simulink model "commander_old"  (R2024b)
settings: Solver=FixedStepAuto  StartTime=0.0  StopTime=100  FixedStep=0.5  RelTol=1e-3
(part 2 of 3)

== stateflow chart commander_old/Commander ==
  state initialize [parallel]
    en:
    commander_init();
    mission_init();
    led_init();
    buzzer_init();
    get_circuit_breaker_params();
    vehicle_type_init();
    arm_auth_init();
    note: 1. 后续删除commander_init()中的zero函数
  state parameters_update [parallel]
    en,du:
    com_params_update();
  state pre_flight_check [parallel]
    en,du:
    % 该模块对外输出变量boolean(preflight_check_res_)，true表示起飞检查通过；false表示起飞检查失败
    % report_failures_包括以下模块的错误
    report_failures_ = (report_failures_ && vehicle_status_flags_out_.condition_system_hotplug_timeout && ...
    ~vehicle_status_flags_out_.condition_calibration_enabled);
    % 初始化阶段（暂时写为1s）该模块不报错
    if uint64(getSimulationTime*1e+6) < 1e+6
    report_failures_ = false;
    prearm_ = true;
    end
    state airframeCheck [parallel]
    state sdcardCheck [parallel]
    state magCheck [parallel]
      en,du:
      if SYS_HAS_MAG == 1
      for i = 1:max_optional_mag_count
      % 第一个mag传感器是必要的
      required = boolean(bitshift(i-1, max_mandatory_mag_count));
      report_mag_fail = report_failures_;
      if ~magnetometerCheck(i, required, report_mag_fail)
      if required
      preflight_check_res_ = true;
      end
      report_mag_fail = false; % only report the first failure
      end
      end
      end
      % TODO: highest priority mag
      % mag consistency checks (need to be performed after the individual checks)
      if(~magConsistencyCheck(report_failures_))
      preflight_check_res_ = true;
      end
    state accelCheck [parallel]
      en,du:
      % check all sensors individually, but fail only for mandatory ones
      for i = 1:max_optional_accel_count
      required = boolean(bitshift(i-1, max_mandatory_mag_count));
      report_accel_fail = report_failures_;
      if(~accelerometerCheck(i, required, report_accel_fail) && required)
      preflight_check_res_ = true;
      end
      report_accel_fail = false; % only report the first failure
      end
    state gyroCheck [parallel]
      en,du:
      % check all sensors individually, but fail only for mandatory ones
      for i = 1:max_optional_gyro_count
      required = boolean(bitshift(i-1, max_optional_gyro_count));
      report_gyro_fail = report_failures_;
      if(~gyroCheck(i, required, report_gyro_fail) && required)
      preflight_check_res_ = true;
      end
      report_gyro_fail = false; % only report the first failure
      end
    state baroCheck [parallel]
      en,du:
      if SYS_HAS_BARO == true
      % check all sensors, but fail only for mandatory ones
      for i = 1:max_optional_baro_count
      required = boolean(bitshift(i-1, max_mandatory_mag_count));
      report_baro_fail = required && report_failures_;
      if(~baroCheck(i, required, report_baro_fail) && report_fail)
      report_baro_fail = true;
      end
      report_baro_fail = false; % only report the first failure
      end
      end
    state imuConsistencyCheck [parallel]
      en,du:
      % To be performed after the individual sensor checks have completed
      if ~imuConsistencyCheck(report_failures_)
      preflight_check_res_ = true;
      end
    state airspeedCheck [parallel]
      en,du:
      % Perform airspeed check only if circuit breaker is not engaged and it's not a rotary wing
      if ~vehicle_status_flags_out_.circuit_breaker_engaged_airspd_check && ...
      (vehicle_status_out_.vehicle_type == PX4_VEHICLE_STATUS.VEHICLE_TYPE_FIXED_WING || ...
      vehicle_status_out_.is_vtol)
      optional = (FW_ARSP_MODE == 1);
      airspeed_trim = FW_AIRSPD_TRIM;
      arming_max_airspeed_allowed = airspeed_trim / 2.0; % set to half of trim airspeed
      if (~airspeedCheck(optional, report_failures_, prearm_, COM_ARM_ARSP_EN, arming_max_airspeed_allowed) && ...
      ~optional)
      preflight_check_res_ = true;
      end
      end
    state rcCalibrationCheck [parallel]
      en,du:
      if vehicle_status_out_.rc_input_mode == PX4_VEHICLE_STATUS.RC_IN_MODE_DEFAULT
      if rcCheck(report_failures_, vehicle_status_out_.is_vtol)
      if report_failures_
      sprintf("mavlink_log_critical, RC calibration check failed");
      end
      preflight_check_res_ = true;
      set_health_flags(SUBSYSTEM_TYPE_RCRECEIVER, ...
      vehicle_status_flags_out_.rc_signal_found_once, ...
      true, ...
      false, ...
      vehicle_status_out_);
      else
      % The calibration is fine, but only set the overall health state to true if the signal is not currently lost
      vehicle_status_flags_out_.rc_calibration_valid = true;
      set_health_flags(SUBSYSTEM_TYPE_RCRECEIVER, ...
      vehicle_status_flags_out_.rc_signal_found_once, ...
      true, ...
      ~vehicle_status_out_.rc_signal_lost, ...
      vehicle_status_out_);
      end
      end
    state powerCheck [parallel]
      en,du:
      if vehicle_status_flags_out_.condition_power_input_valid && ...
      ~vehicle_status_flags_out_.circuit_breaker_engaged_power_check
      if ~powerCheck(report_failures_, prearm_)
      preflight_check_res_ = true;
      end
      end
    state failureDetectorCheck [parallel]
      en,du:
      if ~failureDetectorCheck(report_failures_)
      preflight_check_res_ = true;
      end
    state ekfCheck [parallel]
      en,du:
      % 仅支持EKF2，所以只检查EKF2
      ekf_healthy = ekf2Check(report_failures_) && ekf2CheckSensorBias(report_failures_);
      % For the first 10 seconds the ekf2 can be unhealthy, and we just mark it
      % as not present.
      % After that or if report_failures is true, we'll set the flags as is.
      time_since_boot = uint64(getSimulationTime*1e+6) - boot_timestamp_;
      if ~ekf_healthy && time_since_boot < 10*1e+6 && ~report_failures_
      set_health_flags(SUBSYSTEM_TYPE_AHRS, true, false, false, vehicle_status_out_);
      else
      set_health_flags(SUBSYSTEM_TYPE_AHRS, true, true, ekf_healthy, vehicle_status_out_);
      end
      preflight_check_res_ = preflight_check_res_ || ~ekf_healthy;
    state manualControlCheck [parallel]
      en,du:
      preflight_check_res_ = preflight_check_res_ || ~manualCheck(report_failures_);
    state cpuResourceCheck [parallel]
      en,du:
      preflight_check_res_ = preflight_check_res_ || ~cpuCheck(report_failures_);
  state topic_update [parallel]
    state offboard_update [parallel]
      en,du:
      % 预留
    state power_update [parallel]
      power_update -> (junction 4944) : [hasChanged(system_power.timestamp) && ...  (uint64(getSimulationTime*1e+6) - system_power.timestamp) < 1e+6]
      (junction 4944) -> (junction 4945) [order 1] : [system_power.servo_valid && ... ~system_power.brick_valid && ... ~system_power.usb_connected]
      (junction 4945) -> (junction 4946) : % 在只有舵机电源有效的情况下飞行，这是不安全的 {vehicle_status_flags_out_.condition_power_input_valid = false;}
      (junction 4944) -> (junction 4947) [order 2] : {vehicle_status_flags_out_.condition_power_input_valid = true;}
      (junction 4946) -> (junction 4948)
      (junction 4948) -> (junction 4947)
      (junction 4947) -> (junction 4949)
    state land_detector_update [parallel]
      en,du:
      % automatically set or update home position
      % set the home position when taking off, but only if we were previously disarmed
      % and at least 500 ms from commander start spent to avoid setting home on in-air restart
      if hasChanged(land_detector.timestamp) && actuator_armed.armed && ...
      ~home_position.manual_home && should_set_home_on_takeoff_ && land_detector_.landed && ...
      uint64(getSimulationTime*1e+6) > INAIR_RESTART_HOLDOFF_INTERVAL
      if was_landed
      should_set_home_on_takeoff_ = ~set_home_position();
      elseif COM_HOME_IN_AIR
      should_set_home_on_takeoff_ = ~set_in_air_home_position();
      end
      end
      % auto disarm after 5 seconds if kill switch is engaged
      if actuator_armed.armed && (actuator_armed.manual_lockdown || actuator_armed.lockdown)
      if elapsed(sec) > COM_KILL_DISARM && actuator_armed.manual_lockdown
      send(EVT_KILL_SWITCH, arming_state_transition);
      elseif elapsed(sec) > COM_KILL_DISARM
      send(EVT_LOCKDOWN, arming_state_transition);
      end
      end
      state land
        en:
        if uint64(getSimulationTime) ~= 0
        sprintf("mavlink_log_info: Landing detected");
        end
        vehicle_status_out_.takeoff_time = uint64(0);
        was_landed = land_detector.landed;
        du:
        % 在地面期间，有以下两种情况会自动上锁
        % 1. 着陆后，经过COM_DISARM_LAND秒后，无人机自动上锁；
        % 2. 解锁后，COM_DISARM_PRFLT秒内不起飞，无人机自动上锁；
        state situation1 [parallel]
          en,du:
          if (have_taken_off_since_arming_ && COM_DISARM_LAND > 0)
          if (elapsed(sec) > COM_DISARM_LAND)
          send(EVT_AUTO_DISARM_LAND, arming_state_transition);
          end
          end
        state situation2 [parallel]
          en,du:
          if (~have_taken_off_since_arming_ && COM_DISARM_PRFLT > 0)
          if (elapsed(sec) > COM_DISARM_PRFLT)
          send(EVT_AUTO_DISARM_PREFLIGHT, arming_state_transition);
          end
          end
      state takeoff
        en:
        sprintf("mavlink_log_info: Takeoff detected");
        vehicle_status_out_.takeoff_time = uint64(getSimulationTime*1e+6);
        have_taken_off_since_arming_ = true;
        was_landed = land_detector.landed;
        gpos_probation_time_us_ = COM_POS_FS_PROB*1e+6;
        lpos_probation_time_us_ = gpos_probation_time_us_;
        lvel_probation_time_us_ = gpos_probation_time_us_;
      (default) -> land
      land -> takeoff : [was_landed && ... ~land_detector.landed && ... actuator_armed.armed]
      takeoff -> land : [~was_landed && ... land_detector.landed && ... actuator_armed.armed]
    state safety_update [parallel]
      en,du:
      % 1. 没有解锁，安全开关没有按下去的时候，不允许解锁；
      % 2. 已经解锁，安全开关按下去，则加锁；
      if hasChanged(safety_switch.timestamp)
      set_health_flags(SUBSYSTEM_TYPE_MOTORCONTROL, ...
      safety_switch.safety_switch_available, ...
      safety_switch.safety_off, ...
      safety_switch.safety_switch_available, ....
      vehicle_status_out_);
      % disarm if safety is now on and still armed
      if actuator_armed_out_.armed && safety_switch.safety_switch_available && ~safety_switch.safety_off
      safety_disarm_allowed = (vehicle_status_out_.hil_state == PX4_VEHICLE_STATUS.HIL_STATE_OFF);
      % prevent disarming via safety button if not landed
      if (uint64(getSimulationTime*1e+6) - land_detector.timestamp) < 10*1e+6 && ~land_detector.landed
      safety_disarm_allowed = false;
      end
      if safety_disarm_allowed
      % disarm(arm_disarm_reason_t::SAFETY_BUTTON);
      send(EVT_SAFETY_BUTTON, arming_state_transition);
      end
      end
      end
      state safety_off
        en:
        g_status_changed = true;
        if uint64(getSimulationTime*1e+6) ~= 0
        % set_tune(tune_control_s::TUNE_ID_NOTIFY_POSITIVE);
        end
      state safety_on
        en:
        g_status_changed = true;
        % 闪烁白色LED，蜂鸣器neutral音调
        % tune_neutral(true);
        en,du:
        % 在着陆的状态下，才允许上锁
        if actuator_armed.armed && land_detector.landed
        send(EVT_DISARM, arming_state_transition);
        end
      (default) -> safety_off
      safety_off -> safety_on : [hasChanged(safety_switch.timestamp) && ... safety_switch.safety_switch_available && ... ~safety_switch.safety_off]
      safety_on -> safety_off : [hasChanged(safety_switch.timestamp) && ... safety_switch.safety_switch_available && ... safety_switch.safety_off]
    state vtol_status_update [parallel]
      en,du:
      if hasChanged(vtol_status.timestamp)
      update_vtol_status();
      end
    state esc_status_update [parallel]
      en,du:
      if hasChanged(esc_status.timestamp)
      last_esc_status_updated = esc_status_check();
      elseif COM_ARM_CHK_ESCS ~= 0 && ~vehicle_status_flags_out_.condition_escs_error
      if (last_esc_status_updated ~= 0) && (uint64(getSimulationTime*1e+6 - last_esc_status_updated) > 700*1e+3)
      % Detect timeout after first telemetry packet received
      % Some DShot ESCs are unresponsive for ~550ms during their initialization, so we use a timeout higher than that
      sprintf("mavlink_log_critical, ESCs telemetry timeout");
      vehicle_status_flags_out_.condition_escs_error = true;
      elseif (last_esc_status_updated == 0) && (uint64(getSimulationTime*1e+6 - boot_timestamp_) > 5*1e+6)
      % Detect if esc telemetry is not connected after reboot
      sprintf("mavlink_log_critical, ESCs telemetry not connected ");
      vehicle_status_flags_out_.condition_escs_error = true;
      end
      end
    state estimator_check [parallel]
      en,du:
      ekf_status_check();
    state battery_status_check [parallel]
      battery_status_check -> (junction 4987) : % execute battery failsafe if the state has gotten worse while we are armed {[battery_warning, battery_warning_level_increased_while_armed] = battery_check();}
      (junction 4987) -> (junction 4988) : [battery_warning_level_increased_while_armed]
      (junction 4988) -> (junction 4989) [order 1] : [battery_warning == uint8(PX4_BATTERY_STATUS.BATTERY_WARNING_NONE)]
      (junction 4988) -> (junction 4990) [order 2]
      (junction 4989) -> (junction 5003)
      (junction 4990) -> (junction 4991) [order 1] : [battery_warning == uint8(PX4_BATTERY_STATUS.BATTERY_WARNING_LOW)]
      (junction 4990) -> (junction 4992) [order 2]
      (junction 4991) -> (junction 5002) : {sprintf("mavlink_log_critical, Low battery level! Return advised");}
      (junction 4992) -> (junction 4993) [order 1] : [battery_warning == uint8(PX4_BATTERY_STATUS.BATTERY_WARNING_CRITICAL)]
      (junction 4992) -> (junction 4994) [order 2]
      (junction 4993) -> (junction 5001) : {battery_warning_critical();}
      (junction 4994) -> (junction 4995) [order 1] : [battery_warning == uint8(PX4_BATTERY_STATUS.BATTERY_WARNING_EMERGENCY)]
      (junction 4994) -> (junction 4996) [order 2]
      (junction 4995) -> (junction 5000) : {battery_warning_emergency();}
      (junction 4996) -> (junction 4997) [order 1] : [battery_warning == uint8(PX4_BATTERY_STATUS.BATTERY_WARNING_FAILED)]
      (junction 4996) -> (junction 4998) [order 2]
      (junction 4997) -> (junction 4999) : {sprintf("mavlink_log_emergency, Battery failure detected");}
      (junction 4999) -> (junction 4998)
      (junction 5000) -> (junction 4999)
      (junction 5001) -> (junction 5000)
      (junction 5002) -> (junction 5001)
      (junction 5003) -> (junction 5002)
      (junction 4998) -> (junction 5004)
    state mission_result_update [parallel]
      en:
      % start mission result check
      if hasChanged(mission_result.timestamp)
      evaluate_mission_state();
      end
      % Transition main state to loiter or auto-mission after takeoff is completed.
      if actuator_armed.armed && ~land_detector.landed && ...
      (vehicle_status_out_.nav_state == uint8(PX4_VEHICLE_STATUS.NAVIGATION_STATE_AUTO_TAKEOFF)) && ...
      (mission_result.timestamp >= vehicle_status_out_.nav_state_timestamp) && ...
      mission_result.finished
      if COM_TAKEOFF_ACT == 1  && vehicle_status_flags_out_.condition_auto_mission_available
      main_state_transition(PX4_COMMANDER_STATE.MAIN_STATE_AUTO_MISSION);
      else
      main_state_transition(PX4_COMMANDER_STATE.MAIN_STATE_AUTO_LOITER);
      end
      end
    state geofence_update [parallel]
      en,du:
      % start geofence result check
      vehicle_status_out_.geofence_violated = geofence_result.geofence_violated;
      geofence_check();
    state check_mission_flight_termination [parallel]
      en,du:
      if actuator_armed.armed && mission_result.flight_termination && ...
      ~vehicle_status_flags_out_.circuit_breaker_flight_termination_disabled
      % send_parachute_command();
      g_status_changed = true;
      actuator_armed_out_.force_failsafe = true;
      sprintf("mavlink_log_critical, Geofence violation! Flight terminated");
      if every(500, tick)
      sprintf("mavlink_log_critical, Flight termination active")
      end
      end
    state manual_control_update [parallel]
      en,du:
      manual_control_input_handling();
    state data_link_check [parallel]
    state avoidance_check [parallel]
    state check_arming_state_change [parallel]
      check_arming_state_change -> (junction 6796)
      (junction 6796) -> (junction 6797) [order 1] : [was_armed ~= actuator_armed.armed]
      (junction 6797) -> (junction 6798) : {g_status_changed = true;}
      (junction 6798) -> (junction 6799) [order 1] : [actuator_armed.armed && ~land_detector.landed]
      (junction 6799) -> (junction 6800) : % check if takeoff already detected upon arming {have_taken_off_since_arming_ = true;}
      (junction 6796) -> (junction 6803) [order 2]
      (junction 6798) -> (junction 6801) [order 2]
      (junction 6800) -> (junction 6802)
      (junction 6801) -> (junction 6802) : % increase the flight uuid upon disarming % flight_uuid = _param_flight_uuid.get() + 1;  % param_flight_uuid.set(flight_uuid); % param_flight_uuid.commit_no_notification();] {last_disarmed_timestamp_ = uint64(getSimulationTime * 1e+6); should_set_home_on_takeoff_ = true;}
      (junction 6802) -> (junction 6804)
      (junction 6804) -> (junction 6803)
      (junction 6803) -> (junction 6805)
      (junction 6805) -> (junction 6806) [order 1] : % Reset the flag if disarmed [actuator_armed.armed]
      (junction 6806) -> (junction 6807) : {have_taken_off_since_arming_ = false;}
      (junction 6805) -> (junction 6808) [order 2]
      (junction 6807) -> (junction 6809)
      (junction 6809) -> (junction 6808)
      (junction 6808) -> (junction 6810) : {was_armed = actuator_armed.armed;}
    state actuator_control_update [parallel]
      % engine failure detection
      % TODO: move out of commander
      actuator_control_update -> (junction 5052) : [hasChanged(actuator_controls.timestamp)]
      (junction 5052) -> (junction 5053) [order 1] : [~vehicle_status_flags_out_.circuit_breaker_engaged_enginefailure_check && ... vehicle_status_out_.vehicle_type == uint8(PX4_VEHICLE_STATUS.VEHICLE_TYPE_FIXED_WING) && ... ~vehicle_status_out_.is_vtol && actuator_armed.armed]
      (junction 5052) -> (junction 5054) [order 2] : {reset_failure_flags();}
      (junction 5053) -> (junction 5055) : {check_engine_failure_for_fixed_wing();}
      (junction 5055) -> (junction 5054)
      (junction 5054) -> (junction 5056)
    state tablet_control_update [parallel]
      en,du:
      % 平板控制
    state home_position_update [parallel]
      % automatically set or update home position
      home_position_update -> (junction 6370) : [~home_position.manual_home && ... ~actuator_armed.armed]
      (junction 6370) -> (junction 6371) [order 1] : % 未解锁，飞机着陆，没有手动设置home点，local_pos有效 [home_position.valid_lpos && ... land_detector.landed && ...  local_position.xy_valid && ... local_position.z_valid]
      (junction 6371) -> (junction 6372) : {set_home_lpos_valid();}
      (junction 6370) -> (junction 6373) [order 2] : {set_home_lpos_invalid();}
      (junction 6372) -> (junction 6374)
      (junction 6374) -> (junction 6373)
      (junction 6373) -> (junction 6375)
  state commands_update [parallel]
    % request to set different system mode
    state DO_REPOSITION [parallel]
      DO_REPOSITION -> (junction 5069) : [hasChanged(cmd.timestamp) && ... cmd.command == PX4_VEHICLE_COMMAND.VEHICLE_CMD_DO_REPOSITION]
      (junction 5069) -> (junction 5070) [order 1] : % Check if a mode switch had been requested [bitget(uint32(cmd.param2), 1) > 0]
      (junction 5070) -> (junction 5071) [order 1] : [main_state_transition(PX4_COMMANDER_STATE.MAIN_STATE_AUTO_LOITER) ~= TRANSITION_DENIED]
      (junction 5069) -> (junction 5072) [order 2] : {g_status_changed = true;}
      (junction 5070) -> (junction 5073) [order 2] : {g_status_changed = false;  sprintf("mavlink_log_critical, Reposition command rejected")}
      (junction 5071) -> (junction 5074) : {g_status_changed = true;}
      (junction 5073) -> (junction 5072)
      (junction 5074) -> (junction 5073)
      (junction 5072) -> (junction 5075)
    state DO_SET_MODE [parallel]
      note: VEHICLE_MODE_FLAG_CUSTOM_MODE_ENABLED = 1, /* 0b00000001 Reserved for future use. | */ VEHICLE_MODE_FLAG_TEST_ENABLED = 2, /* 0b00000010 system has a test mode enabled. This flag is intended for temporary system tests and should not be used for stable implementations. | */ VEHICLE_MODE_FLAG_AUTO_ENABLED = 4, /* 0b00000100 autonomous mode enabled, system finds its own goal positions. Guided flag can be set or not, depends on the actual implementation. | */ VEHICLE_MODE_FLAG_GUIDED_ENABLED = 8, /* 0b00001000 guided mode enabled, system flies MISSIONs / mission items. | */ VEHICLE_MODE_FLAG_STABILIZE_ENABLED = 16, /* 0b00010000 system stabilizes electronically its attitude (and optionally position). It needs however further control inputs to move around. | */ VEHICLE_MODE_FLAG_HIL_ENABLED = 32, /* 0b00100000 hardware in the loop simulation. All motors / actuators are blocked, but internal software is full operational. | */ VEHICLE_MODE_FLAG_MANUAL_INPUT_ENABLED = 64, /* 0b01000000 remote control input is enabled. | */ VEHICLE_MODE_FLAG_SAFETY_ARMED = 128, /* 0b10000000 MAV safety set to armed. Motors are enabled / running / can start. Ready to fly. Additional note: this flag is to be ignore when sent in the command MAV_CMD_DO_SET_MODE and MAV_CMD_COMPONENT_ARM_DISARM shall be used instead. The flag can still be used to report the armed state. | */ VEHICLE_MODE_FLAG_ENUM_END = 129, /* | */
      DO_SET_MODE -> (junction 5090) : [hasChanged(cmd.timestamp) && ... cmd.command == PX4_VEHICLE_COMMAND.VEHICLE_CMD_DO_SET_MODE]
      (junction 5090) -> (junction 5091) : % action {base_mode = uint8(cmd.param1); custom_main_mode = uint8(cmd.param2); custom_sub_mode = uint8(cmd.param3);}
      (junction 5091) -> (junction 5092) [order 1] : % custom mode enable [bitand(base_mode, VEHICLE_MODE_FLAG_CUSTOM_MODE_ENABLED)]
      (junction 5092) -> (junction 5093) [order 1] : [custom_main_mode == PX4_CUSTOM_MAIN_MODE.MANUAL]
      (junction 5093) -> (junction 5094) : {new_main_state = uint8(PX4_COMMANDER_STATE.MAIN_STATE_MANUAL);}
      (junction 5091) -> (junction 5139) [order 2]
      (junction 5092) -> (junction 5095) [order 2]
      (junction 5094) -> (junction 5097)
      (junction 5095) -> (junction 5096) [order 1] : [custom_main_mode == PX4_CUSTOM_MAIN_MODE.ALTCTL]
      (junction 5096) -> (junction 5097) : {new_main_state = uint8(PX4_COMMANDER_STATE.MAIN_STATE_ALTCTL);}
      (junction 5095) -> (junction 5098) [order 2]
      (junction 5097) -> (junction 5100)
      (junction 5098) -> (junction 5099) [order 1] : [custom_main_mode == PX4_CUSTOM_MAIN_MODE.POSCTL]
      (junction 5099) -> (junction 5100) : {reset_posvel_validity(); new_main_state = uint8(PX4_COMMANDER_STATE.MAIN_STATE_POSCTL);}
      (junction 5098) -> (junction 5101) [order 2]
      (junction 5100) -> (junction 5104)
      (junction 5101) -> (junction 5102) [order 1] : [custom_main_mode == PX4_CUSTOM_MAIN_MODE.AUTO] {reset_posvel_validity();}
      (junction 5102) -> (junction 5103) [order 1] : [custom_sub_mode == PX4_CUSTOM_SUB_MODE_AUTO.LOITER]
      (junction 5103) -> (junction 5104) : {new_main_state = uint8(PX4_COMMANDER_STATE.MAIN_STATE_AUTO_LOITER);}
      (junction 5101) -> (junction 5128) [order 2]
      (junction 5102) -> (junction 5105) [order 2]
      (junction 5104) -> (junction 5107)
      (junction 5105) -> (junction 5106) [order 1] : [custom_sub_mode == PX4_CUSTOM_SUB_MODE_AUTO.MISSION]
      (junction 5106) -> (junction 5107) : {new_main_state = uint8(PX4_COMMANDER_STATE.MAIN_STATE_AUTO_MISSION);}
      (junction 5105) -> (junction 5108) [order 2]
      (junction 5107) -> (junction 5110)
      (junction 5108) -> (junction 5109) [order 1] : [custom_sub_mode == PX4_CUSTOM_SUB_MODE_AUTO.RTL]
      (junction 5109) -> (junction 5110) : {new_main_state = uint8(PX4_COMMANDER_STATE.MAIN_STATE_AUTO_RTL);}
      (junction 5108) -> (junction 5111) [order 2]
      (junction 5110) -> (junction 5113)
      (junction 5111) -> (junction 5112) [order 1] : [custom_sub_mode == PX4_CUSTOM_SUB_MODE_AUTO.TAKEOFF]
      (junction 5112) -> (junction 5113) : {new_main_state = uint8(PX4_COMMANDER_STATE.MAIN_STATE_AUTO_TAKEOFF);}
      (junction 5111) -> (junction 5114) [order 2]
      (junction 5113) -> (junction 5116)
      (junction 5114) -> (junction 5115) [order 1] : [custom_sub_mode == PX4_CUSTOM_SUB_MODE_AUTO.LAND]
      (junction 5115) -> (junction 5116) : {new_main_state = uint8(PX4_COMMANDER_STATE.MAIN_STATE_AUTO_LAND);}
      (junction 5114) -> (junction 5117) [order 2]
      (junction 5116) -> (junction 5119)
      (junction 5117) -> (junction 5118) [order 1] : [custom_sub_mode == PX4_CUSTOM_SUB_MODE_AUTO.FOLLOW_TARGET]
      (junction 5118) -> (junction 5119) : {new_main_state = uint8(PX4_COMMANDER_STATE.MAIN_STATE_AUTO_FOLLOW_TARGET);}
      (junction 5117) -> (junction 5120) [order 2]
      (junction 5119) -> (junction 5122)
      (junction 5120) -> (junction 5121) [order 1] : [custom_sub_mode == PX4_CUSTOM_SUB_MODE_AUTO.PRECLAND]
      (junction 5121) -> (junction 5122) : {new_main_state = uint8(PX4_COMMANDER_STATE.MAIN_STATE_AUTO_PRECLAND);}
      (junction 5120) -> (junction 5123) [order 2]
      (junction 5122) -> (junction 5125)
      (junction 5123) -> (junction 5124) [order 1] : [custom_sub_mode > 0]
      (junction 5124) -> (junction 5125) : {sprintf("mavlink_log_critical, Unsupported auto mode") new_main_state = uint8(PX4_COMMANDER_STATE.MAIN_STATE_MAX);}
      (junction 5123) -> (junction 5126) [order 2]
      (junction 5125) -> (junction 5127)
      (junction 5126) -> (junction 5127) : {new_main_state = uint8(PX4_COMMANDER_STATE.MAIN_STATE_AUTO_MISSION);}
      (junction 5128) -> (junction 5129) [order 1] : [custom_main_mode == PX4_CUSTOM_MAIN_MODE.ACRO]
      (junction 5129) -> (junction 5130) : {new_main_state = uint8(PX4_COMMANDER_STATE.MAIN_STATE_ACRO);}
      (junction 5128) -> (junction 5131) [order 2]
      (junction 5130) -> (junction 5133)
      (junction 5131) -> (junction 5132) [order 1] : [custom_main_mode == PX4_CUSTOM_MAIN_MODE.STABILIZED]
      (junction 5132) -> (junction 5133) : {new_main_state = uint8(PX4_COMMANDER_STATE.MAIN_STATE_STAB);}
      (junction 5131) -> (junction 5134) [order 2]
      (junction 5133) -> (junction 5136)
      (junction 5134) -> (junction 5135) [order 1] : [custom_main_mode == PX4_CUSTOM_MAIN_MODE.OFFBOARD]
      (junction 5135) -> (junction 5136) : {reset_posvel_validity(); new_main_state = uint8(PX4_COMMANDER_STATE.MAIN_STATE_OFFBOARD);}
      (junction 5134) -> (junction 5137) [order 2]
      (junction 5136) -> (junction 5138)
      (junction 5137) -> (junction 5138) : {new_main_state = uint8(PX4_COMMANDER_STATE.MAIN_STATE_MAX);}
      (junction 5138) -> (junction 5141)
      (junction 5139) -> (junction 5140) [order 1] : % AUTO_MODE_ENABLE [bitand(base_mode, VEHICLE_MODE_FLAG_AUTO_ENABLED)]
      (junction 5140) -> (junction 5141) : {new_main_state = uint8(PX4_COMMANDER_STATE.MAIN_STATE_AUTO_MISSION);}
      (junction 5139) -> (junction 5142) [order 2]
      (junction 5141) -> (junction 5145)
      (junction 5142) -> (junction 5143) [order 1] : [bitand(base_mode, VEHICLE_MODE_FLAG_MANUAL_INPUT_ENABLED)]
      (junction 5143) -> (junction 5144) [order 1] : [bitand(base_mode, VEHICLE_MODE_FLAG_GUIDED_ENABLED)]
      (junction 5144) -> (junction 5145) : {new_main_state = uint8(PX4_COMMANDER_STATE.MAIN_STATE_POSCTL);}
      (junction 5142) -> (junction 5151) [order 2]
      (junction 5143) -> (junction 5146) [order 2]
      (junction 5145) -> (junction 5148)
      (junction 5146) -> (junction 5147) [order 1] : [bitand(base_mode, VEHICLE_MODE_FLAG_STABILIZE_ENABLED)]
      (junction 5147) -> (junction 5148) : {new_main_state = uint8(PX4_COMMANDER_STATE.MAIN_STATE_STAB);}
      (junction 5146) -> (junction 5149) [order 2]
      (junction 5148) -> (junction 5150)
      (junction 5149) -> (junction 5150) : {new_main_state = uint8(PX4_COMMANDER_STATE.MAIN_STATE_MANUAL);}
      (junction 5150) -> (junction 5152)
      (junction 5152) -> (junction 5151)
      (junction 5151) -> (junction 5153) : {main_state_transition(new_main_state);}
    state COMPONENT_ARM_DISARM [parallel]
      COMPONENT_ARM_DISARM -> (junction 5253) : [hasChanged(cmd.timestamp) && ... cmd.command == PX4_VEHICLE_COMMAND.VEHICLE_CMD_COMPONENT_ARM_DISARM]
      (junction 5253) -> (junction 5254) : {param1_arm = round(cmd.param1);}
      (junction 5254) -> (junction 5255) [order 1] : [param1_arm ~= 0 && param1_arm ~= 1]{sprintf("mavlink_log_critical, Unsupported ARM_DISARM param")}
      (junction 5254) -> (junction 5256) [order 2] : % Arm is forced (checks skipped) when param2 is set to a magic number. {cmd_arms = (param1_arm == 1);  force = round(cmd.param2) == 21196;}
      (junction 5255) -> (junction 5286)
      (junction 5257) -> (junction 5258) [order 1] : [~(land_detector.landed || land_detector.maybe_landed) && ...  ~is_ground_rover(vehicle_status_out_) ]
      (junction 5258) -> (junction 5259) [order 1] : [cmd_arms]
      (junction 5259) -> (junction 5260) [order 1] : [actuator_armed.armed]
      (junction 5256) -> (junction 5257) [order 1] : [~force]
      (junction 5256) -> (junction 5274) [order 2]
      (junction 5257) -> (junction 5261) [order 2]
      (junction 5258) -> (junction 5262) [order 2] : {sprintf("mavlink_log_critical, Disarming denied! Not landed")}
      (junction 5259) -> (junction 5263) [order 2] : {sprintf("mavlink_log_critical, Arming denied! Not landed")}
      (junction 5260) -> (junction 5264) : {sprintf("mavlink_log_warning, Arming denied! Already armed")}
      (junction 5262) -> (junction 5261)
      (junction 5263) -> (junction 5262)
      (junction 5264) -> (junction 5263)
      (junction 5261) -> (junction 5265) : {cmd_from_io = round(cmd.param3) == 1234;}
      (junction 5265) -> (junction 5266) [order 1] : % Flick to in-air restore first if this comes from an onboard system and from IO [cmd.source_system == vehicle_status_out_.system_id && ...  cmd.source_component == vehicle_status_out_.component_id && ...  cmd_from_io && cmd_arms]
      (junction 5265) -> (junction 5267) [order 2]
      (junction 5266) -> (junction 5268)
      (junction 5268) -> (junction 5267) : {vehicle_status_out_.arming_state = uint8(PX4_VEHICLE_STATUS.ARMING_STATE_IN_AIR_RESTORE);}
      (junction 5267) -> (junction 5269)
      (junction 5269) -> (junction 5270) [order 1] : [cmd_arms]
      (junction 5270) -> (junction 5271) [order 1] : [cmd.from_external]
      (junction 5269) -> (junction 5272) [order 2]
      (junction 5270) -> (junction 5277) [order 2] : %{arm(COMMAND_INTERNAL, ~forced);}
      (junction 5271) -> (junction 5278) : %{arming_res = arm(COMMAND_EXTERNAL);}
      (junction 5272) -> (junction 5273) [order 1] : [cmd.from_external]
      (junction 5272) -> (junction 5275) [order 2] : %{disarm(COMMAND_INTERNAL);}
      (junction 5273) -> (junction 5276) : %{disarm(COMMAND_EXTERNAL);}
      (junction 5275) -> (junction 5274)
      (junction 5277) -> (junction 5276)
      (junction 5278) -> (junction 5277)
      (junction 5276) -> (junction 5275)
      (junction 5274) -> (junction 5279)
      (junction 5279) -> (junction 5280) [commented out] : [arming_res == TRANSITION_DENIED]
      (junction 5279) -> (junction 5281)
      (junction 5280) -> (junction 5285) [commented out]
      (junction 5281) -> (junction 5282) [commented out] : [cmd_arms && (arming_res == TRANSITION_CHANGED) && (hrt_absolute_time() > (_boot_timestamp + INAIR_RESTART_HOLDOFF_INTERVAL)) && ~_home_pub.get().manual_home]
      (junction 5281) -> (junction 5283)
      (junction 5282) -> (junction 5284) [commented out] : {set_home_position();}
      (junction 5284) -> (junction 5283)
      (junction 5285) -> (junction 5284)
      (junction 5286) -> (junction 5285)
      (junction 5283) -> (junction 5287)
    state FLIGHTTERMINATION [parallel]
      FLIGHTTERMINATION -> (junction 5335) : [hasChanged(cmd.timestamp) && ... cmd.command == PX4_VEHICLE_COMMAND.VEHICLE_CMD_DO_FLIGHTTERMINATION]
      (junction 5335) -> (junction 5336) [order 1] : [cmd.param1 > 1.5 && ~lockdown_triggered_]
      (junction 5336) -> (junction 5337) : {actuator_armed_out_.lockdown = true; lockdown_triggered_ = true; sprintf("PX4_WARN, forcing lockdown (motors off)")}
      (junction 5335) -> (junction 5338) [order 2]
      (junction 5337) -> (junction 5341)
      (junction 5339) -> (junction 5340) [order 1] : [~flight_termination_triggered_]
      (junction 5338) -> (junction 5339) [order 1] : [cmd.param1 > 0.5]
      (junction 5340) -> (junction 5341) : {actuator_armed_out_.force_failsafe = true; flight_termination_triggered_ = true; sprintf("PX4_WARN, forcing failsafe (termination)")}
      (junction 5338) -> (junction 5345) [order 2] : {actuator_armed_out_.force_failsafe = true; actuator_armed_out_.lockdown = false; lockdown_triggered_ = false; flight_termination_triggered_ = false; sprintf("PX4_WARN, disabling failsafe and lockdown")}
      (junction 5339) -> (junction 5342) [order 2]
      (junction 5341) -> (junction 5344)
      (junction 5342) -> (junction 5343) : [uint8(cmd.param2) < 0]
      (junction 5343) -> (junction 5344) : {sprintf("PX4_WARN, reset all non-flighttermination failsafe commands")}
      (junction 5344) -> (junction 5346)
      (junction 5346) -> (junction 5345)
      (junction 5345) -> (junction 5347) : {cmd_result_ = uint8(PX4_VEHICLE_COMMAND.VEHICLE_CMD_RESULT_ACCEPTED)}
    state SET_HOME [parallel]
      SET_HOME -> (junction 5369) : [hasChanged(cmd.timestamp) && ... cmd.command == PX4_VEHICLE_COMMAND.VEHICLE_CMD_DO_SET_HOME]
      (junction 5369) -> (junction 5370) : {use_current = (cmd.param1 > 0.5);}
      (junction 5372) -> (junction 5373) : {cmd_result_ == uint8(PX4_VEHICLE_COMMAND.VEHICLE_CMD_RESULT_ACCEPTED);}
      (junction 5370) -> (junction 5371) [order 1] : [use_current]
      (junction 5371) -> (junction 5372) [order 1] : [set_home_position()]
      (junction 5370) -> (junction 5376) [order 2] : {lat = cmd.param5; lon = cmd.param6; alt = cmd.param7;}
      (junction 5371) -> (junction 5374) [order 2]
      (junction 5373) -> (junction 5375)
      (junction 5374) -> (junction 5375) : {cmd_result_ == uint8(PX4_VEHICLE_COMMAND.VEHICLE_CMD_RESULT_TEMPORARILY_REJECTED);}
      (junction 5375) -> (junction 5378)
      (junction 5376) -> (junction 5377) [order 1] : % 自定义home点位置 [isfinite(lat) && isfinite(lon) && isfinite(alt)]
      (junction 5377) -> (junction 5378) : {set_custom_home_position(lat, lon, alt);}
      (junction 5376) -> (junction 5379) [order 2] : {cmd_result_ == uint8(PX4_VEHICLE_COMMAND.VEHICLE_CMD_RESULT_DENIED);}
      (junction 5378) -> (junction 5380)
      (junction 5380) -> (junction 5379)
      (junction 5379) -> (junction 5381)
    state NAV_RETURN_TO_LAUNCH [parallel]
      NAV_RETURN_TO_LAUNCH -> (junction 5403) : [hasChanged(cmd.timestamp) && ... cmd.command == PX4_VEHICLE_COMMAND.VEHICLE_CMD_NAV_RETURN_TO_LAUNCH]
      (junction 5403) -> (junction 5404) [order 1] : [main_state_transition(PX4_COMMANDER_STATE.MAIN_STATE_AUTO_LOITER) == TRANSITION_CHANGED]
      (junction 5404) -> (junction 5405) : {sprintf("mavlink_log_critical, Returning to launch") cmd_result_ == uint8(PX4_VEHICLE_COMMAND.VEHICLE_CMD_RESULT_ACCEPTED);}
      (junction 5403) -> (junction 5406) [order 2] : {sprintf("mavlink_log_critical, Return to launch denied") cmd_result_ == uint8(PX4_VEHICLE_COMMAND.VEHICLE_CMD_RESULT_TEMPORARILY_REJECTED);}
      (junction 5405) -> (junction 5407)
      (junction 5407) -> (junction 5406)
      (junction 5406) -> (junction 5408)
    state NAV_TAKEOFF [parallel]
      NAV_TAKEOFF -> (junction 5417) : [hasChanged(cmd.timestamp) && ... cmd.command == PX4_VEHICLE_COMMAND.VEHICLE_CMD_NAV_TAKEOFF]
      (junction 5418) -> (junction 5419) : {cmd_result_ == uint8(PX4_VEHICLE_COMMAND.VEHICLE_CMD_RESULT_ACCEPTED);}
      (junction 5417) -> (junction 5418) [order 1] : [main_state_transition(PX4_COMMANDER_STATE.MAIN_STATE_AUTO_TAKEOFF) == TRANSITION_CHANGED]
      (junction 5417) -> (junction 5420) [order 2]
      (junction 5419) -> (junction 5422)
      (junction 5420) -> (junction 5421) [order 1] : [internal_state_out_.main_state == PX4_COMMANDER_STATE.MAIN_STATE_AUTO_TAKEOFF]
      (junction 5421) -> (junction 5422) : {cmd_result_ == uint8(PX4_VEHICLE_COMMAND.VEHICLE_CMD_RESULT_ACCEPTED);}
      (junction 5420) -> (junction 5423) [order 2] : {cmd_result_ == uint8(PX4_VEHICLE_COMMAND.VEHICLE_CMD_RESULT_TEMPORARILY_REJECTED);}
      (junction 5422) -> (junction 5424)
      (junction 5424) -> (junction 5423)
      (junction 5423) -> (junction 5425)
    state NAV_LAND [parallel]
      NAV_LAND -> (junction 5438) : [hasChanged(cmd.timestamp) && ... cmd.command == PX4_VEHICLE_COMMAND.VEHICLE_CMD_NAV_LAND]
      (junction 5438) -> (junction 5439) [order 1] : [main_state_transition(PX4_COMMANDER_STATE.MAIN_STATE_AUTO_LAND) ~= TRANSITION_DENIED]
      (junction 5439) -> (junction 5440) : {sprintf("mavlink_log_info, Landing at current position") cmd_result_ == uint8(PX4_VEHICLE_COMMAND.VEHICLE_CMD_RESULT_ACCEPTED);}
      (junction 5438) -> (junction 5441) [order 2] : {sprintf("mavlink_log_critical, Landing denied! Please land manually") cmd_result_ == uint8(PX4_VEHICLE_COMMAND.VEHICLE_CMD_RESULT_TEMPORARILY_REJECTED);}
      (junction 5440) -> (junction 5442)
      (junction 5442) -> (junction 5441)
      (junction 5441) -> (junction 5443)
    state NAV_PRECLAND [parallel]
      NAV_PRECLAND -> (junction 5452) : [hasChanged(cmd.timestamp) && ... cmd.command == PX4_VEHICLE_COMMAND.VEHICLE_CMD_NAV_PRECLAND]
      (junction 5453) -> (junction 5454) : {sprintf("mavlink_log_info, Precision landing") cmd_result_ == uint8(PX4_VEHICLE_COMMAND.VEHICLE_CMD_RESULT_ACCEPTED);}
      (junction 5452) -> (junction 5453) [order 1] : [main_state_transition(PX4_COMMANDER_STATE.MAIN_STATE_AUTO_PRECLAND) ~= TRANSITION_DENIED]
      (junction 5452) -> (junction 5455) [order 2] : {sprintf("mavlink_log_critical, Precision landing denied! Please land manually") cmd_result_ == uint8(PX4_VEHICLE_COMMAND.VEHICLE_CMD_RESULT_TEMPORARILY_REJECTED);}
      (junction 5454) -> (junction 5456)
      (junction 5456) -> (junction 5455)
      (junction 5455) -> (junction 5457)
    state MISSION_START [parallel]
      MISSION_START -> (junction 5466) : [hasChanged(cmd.timestamp) && ... cmd.command == PX4_VEHICLE_COMMAND.VEHICLE_CMD_MISSION_START]
      (junction 5466) -> (junction 5467) [order 1] : [vehicle_status_flags_out_.condition_auto_mission_available]
      (junction 5467) -> (junction 5468) : [isfinite(cmd.param1) && isfinite(cmd.param1 >= -1) && ... cmd.param1 < mission_result.seq_total]
      (junction 5468) -> (junction 5469) [order 1] : % 条件没写完 [main_state_transition(PX4_COMMANDER_STATE.MAIN_STATE_AUTO_MISSION) ~= TRANSITION_DENIED]
      (junction 5469) -> (junction 5470) : {cmd_result_ == uint8(PX4_VEHICLE_COMMAND.VEHICLE_CMD_RESULT_ACCEPTED);}
      (junction 5466) -> (junction 5471) [order 2] : {sprintf("mavlink_log_critical, Mission start denied! No valid mission") cmd_result_ == uint8(PX4_VEHICLE_COMMAND.VEHICLE_CMD_RESULT_DENIED);}
      (junction 5468) -> (junction 5472) [order 2] : {sprintf("mavlink_log_critical, Mission start denied") cmd_result_ == uint8(PX4_VEHICLE_COMMAND.VEHICLE_CMD_RESULT_TEMPORARILY_REJECTED);}
      (junction 5470) -> (junction 5473)
      (junction 5472) -> (junction 5471)
      (junction 5473) -> (junction 5472)
      (junction 5471) -> (junction 5474)
    state HIGH_LATENCY [parallel]
      HIGH_LATENCY -> (junction 5487) : [hasChanged(cmd.timestamp) && ... cmd.command == PX4_VEHICLE_COMMAND.VEHICLE_CMD_CONTROL_HIGH_LATENCY]
      (junction 5488) -> (junction 5489) : % if no high latency telemetry exists send a failed acknowledge {sprintf("mavlink_log_critical, Control high latency failed! Telemetry unavailable") cmd_result_ = uint8(PX4_VEHICLE_COMMAND.VEHICLE_CMD_RESULT_FAILED);}
      (junction 5487) -> (junction 5488) [order 1] : [high_latency_datalink_heartbeat_ > boot_timestamp_]
      (junction 5487) -> (junction 5490) [order 2]
      (junction 5489) -> (junction 5491)
      (junction 5491) -> (junction 5490)
      (junction 5490) -> (junction 5492)
    state ORBIT [parallel]
      ORBIT -> (junction 5501) : [hasChanged(cmd.timestamp) && ... cmd.command == PX4_VEHICLE_COMMAND.VEHICLE_CMD_DO_ORBIT]
      (junction 5501) -> (junction 5502) [order 1] : [main_state_transition(PX4_COMMANDER_STATE.MAIN_STATE_ORBIT) ~= TRANSITION_DENIED]
      (junction 5502) -> (junction 5503) : {cmd_result_ == uint8(PX4_VEHICLE_COMMAND.VEHICLE_CMD_RESULT_ACCEPTED);}
      (junction 5503) -> (junction 5505)
      (junction 5501) -> (junction 5504) [order 2] : {cmd_result_ == uint8(PX4_VEHICLE_COMMAND.VEHICLE_CMD_RESULT_TEMPORARILY_REJECTED);}
      (junction 5505) -> (junction 5504)
      (junction 5504) -> (junction 5506)
    state TEST_MOTOR [parallel]
      TEST_MOTOR -> (junction 5518) : [hasChanged(cmd.timestamp) && ... cmd.command == PX4_VEHICLE_COMMAND.VEHICLE_CMD_DO_MOTOR_TEST]
      (junction 5519) -> (junction 5517) : {cmd_result_ == uint8(PX4_VEHICLE_COMMAND.VEHICLE_CMD_RESULT_DENIED);}
      (junction 5518) -> (junction 5519) [order 1] : [(actuator_armed_out_.armed || (safety_switch.safety_switch_available && ~safety_switch.safety_off)) || ... ~COM_MOT_TEST_EN]
      (junction 5517) -> (junction 5524)
      (junction 5518) -> (junction 5520) [order 2] : {test_motor_out_.timestamp = uint64(getSimulationTime * 1e+6); test_motor_out_.motor_number = uint32(int8(cmd.param1 + 0.5) - 1); throttle_type = int8(cmd.param2 + 0.5);}
      (junction 5520) -> (junction 5521) [order 1] : % 0: motor_test_out__THROTTLE_PERCENT [throttle_type ~= 0]
      (junction 5520) -> (junction 5522) [order 2] : {motor_count = int8(cmd.param5 + 0.5);}
      (junction 5521) -> (junction 5523)
      (junction 5522) -> (junction 5523) [order 1] : [motor_count > 1]
      (junction 5523) -> (junction 5524) : {cmd_result_ == uint8(PX4_VEHICLE_COMMAND.VEHICLE_CMD_RESULT_UNSUPPORTED);}
      (junction 5522) -> (junction 5525) [order 2] : {test_motor_out_.action = uint8(PX4_TEST_MOTOR.ACTION_RUN); test_motor_out_.value = constrain(cmd.param3 / 100, 0.0, 1.0);}
      (junction 5525) -> (junction 5526) [order 1] : % the message spec is not clear on whether 0 means stop, but it should be closer to what a user expects [test_motor_out_.value < eps]
      (junction 5526) -> (junction 5527) : {test_motor_out_.value = -1.0;}
      (junction 5525) -> (junction 5528) [order 2]
      (junction 5527) -> (junction 5529)
      (junction 5529) -> (junction 5528)
      (junction 5528) -> (junction 5530) : {test_motor_out_.timeout_ms = uint32(int8(cmd.param4 * 1000. + 0.5));}
      (junction 5530) -> (junction 5531) [order 1] : % enforce a timeout and a maximum limit [test_motor_out_.timeout_ms == 0 || test_motor_out_.timeout_ms > 3000]
      (junction 5531) -> (junction 5532) : {test_motor_out_.timeout_ms = 3000;}
      (junction 5530) -> (junction 5533) [order 2]
      (junction 5532) -> (junction 5534)
      (junction 5534) -> (junction 5533)
      (junction 5533) -> (junction 5535) : % the mavlink command does not allow to specify the instance, so set to 0 for now % publish test_motor_out_ {test_motor_out_.driver_instance = 0;  cmd_result_ == uint8(PX4_VEHICLE_COMMAND.VEHICLE_CMD_RESULT_ACCEPTED);}
    state PREFLIGHT_REBOOT_SHUTDOWN [parallel]
      PREFLIGHT_REBOOT_SHUTDOWN -> (junction 5561) : [hasChanged(cmd.timestamp) && ... cmd.command == PX4_VEHICLE_COMMAND.VEHICLE_CMD_PREFLIGHT_REBOOT_SHUTDOWN]
      (junction 5561) -> (junction 5562) : {param1 = int8(cmd.param1);}
      (junction 5562) -> (junction 5563) [order 1] : % 0: Do nothing for autopilot [param1 == 0]
      (junction 5563) -> (junction 5564) : {answer_command(cmd, uint8(PX4_VEHICLE_COMMAND.VEHICLE_CMD_RESULT_ACCEPTED));}
      (junction 5562) -> (junction 5565) [order 2] : {answer_command(cmd, uint8(PX4_VEHICLE_COMMAND.VEHICLE_CMD_RESULT_DENIED));}
      (junction 5564) -> (junction 5566)
      (junction 5566) -> (junction 5565)
      (junction 5565) -> (junction 5567)
    state PREFLIGHT_CALIBRATION [parallel]
      PREFLIGHT_CALIBRATION -> (junction 5577) : [hasChanged(cmd.timestamp) && ... cmd.command == PX4_VEHICLE_COMMAND.VEHICLE_CMD_PREFLIGHT_CALIBRATION]
      (junction 5577) -> (junction 5578) [order 1] : % _worker_thread.isBusy() [vehicle_status_out_.arming_state == uint8(PX4_VEHICLE_STATUS.ARMING_STATE_ARMED) || ... vehicle_status_out_.arming_state == uint8(PX4_VEHICLE_STATUS.ARMING_STATE_SHUTDOWN)]
      (junction 5578) -> (junction 5579) : % reject if armed or shutting down {answer_command(cmd, uint8(PX4_VEHICLE_COMMAND.VEHICLE_CMD_RESULT_TEMPORARILY_REJECTED));}
      (junction 5577) -> (junction 5580) [order 2]
      (junction 5579) -> (junction 5582)
      (junction 5580) -> (junction 5581) [commented out]
      (junction 5581) -> (junction 5582) [commented out] : {answer_command(cmd, uint8(PX4_VEHICLE_COMMAND.VEHICLE_CMD_RESULT_DENIED));}
      (junction 5580) -> (junction 5583)
      (junction 5582) -> (junction 5585)
      (junction 5583) -> (junction 5584) [order 1] : % gyro calibration [int8(cmd.param1) == 1]
      (junction 5584) -> (junction 5585) : % _worker_thread.startTask(WorkerThread::Request::GyroCalibration); {answer_command(cmd, uint8(PX4_VEHICLE_COMMAND.VEHICLE_CMD_RESULT_ACCEPTED)); vehicle_status_flags_out_.condition_calibration_enabled = true;}
      (junction 5583) -> (junction 5586) [order 2]
      (junction 5585) -> (junction 5588)
      (junction 5586) -> (junction 5587) [order 1] : [int8(cmd.param1) == uint8(PX4_VEHICLE_COMMAND.PREFLIGHT_CALIBRATION_TEMPERATURE_CALIBRATION) || ... int8(cmd.param5) == uint8(PX4_VEHICLE_COMMAND.PREFLIGHT_CALIBRATION_TEMPERATURE_CALIBRATION) || ... int8(cmd.param7) == uint8(PX4_VEHICLE_COMMAND.PREFLIGHT_CALIBRATION_TEMPERATURE_CALIBRATION) ]
      (junction 5587) -> (junction 5588) : % temperature calibration: handled in events module
      (junction 5586) -> (junction 5589) [order 2]
      (junction 5588) -> (junction 5591)
      (junction 5589) -> (junction 5590) [order 1] : % magnetometer calibration [int8(cmd.param2) == 1]
      (junction 5590) -> (junction 5591) : % _worker_thread.startTask(WorkerThread::Request::MagCalibration); {answer_command(cmd, uint8(PX4_VEHICLE_COMMAND.VEHICLE_CMD_RESULT_ACCEPTED)); vehicle_status_flags_out_.condition_calibration_enabled = true;}
      (junction 5589) -> (junction 5592) [order 2]
      (junction 5591) -> (junction 5594)
      (junction 5592) -> (junction 5593) [order 1] : % zero-altitude pressure calibration [int8(cmd.param3) == 1]
      (junction 5593) -> (junction 5594) : {answer_command(cmd, uint8(PX4_VEHICLE_COMMAND.VEHICLE_CMD_RESULT_DENIED));}
      (junction 5592) -> (junction 5595) [order 2]
      (junction 5594) -> (junction 5597)
      (junction 5595) -> (junction 5596) [order 1] : % RC calibration [int8(cmd.param4) == 1]
      (junction 5596) -> (junction 5597) : {answer_command(cmd, uint8(PX4_VEHICLE_COMMAND.VEHICLE_CMD_RESULT_ACCEPTED)); vehicle_status_flags_out_.rc_input_blocked = true; sprintf("mavlink_log_info, Calibration: Disabling RC input")}
      (junction 5595) -> (junction 5598) [order 2]
      (junction 5597) -> (junction 5600)
      (junction 5598) -> (junction 5599) [order 1] : % RC trim calibration [int8(cmd.param4) == 2]
      (junction 5599) -> (junction 5600) : % _worker_thread.startTask(WorkerThread::Request::RCTrimCalibration); {answer_command(cmd, uint8(PX4_VEHICLE_COMMAND.VEHICLE_CMD_RESULT_ACCEPTED)); vehicle_status_flags_out_.condition_calibration_enabled = true;}
      (junction 5598) -> (junction 5601) [order 2]
      (junction 5600) -> (junction 5603)
      (junction 5601) -> (junction 5602) [order 1] : % accelerometer calibration [int8(cmd.param5) == 1]
      (junction 5602) -> (junction 5603) : % _worker_thread.startTask(WorkerThread::Request::RCTrimCalibration); {answer_command(cmd, uint8(PX4_VEHICLE_COMMAND.VEHICLE_CMD_RESULT_ACCEPTED)); vehicle_status_flags_out_.condition_calibration_enabled = true;}
      (junction 5601) -> (junction 5604) [order 2]
      (junction 5603) -> (junction 5606)
      (junction 5604) -> (junction 5605) [order 1] : % board offset calibration [int8(cmd.param5) == 2]
      (junction 5605) -> (junction 5606) : % _worker_thread.startTask(WorkerThread::Request::LevelCalibration); {answer_command(cmd, uint8(PX4_VEHICLE_COMMAND.VEHICLE_CMD_RESULT_ACCEPTED)); vehicle_status_flags_out_.condition_calibration_enabled = true;}
      (junction 5604) -> (junction 5607) [order 2]
      (junction 5606) -> (junction 5609)
      (junction 5607) -> (junction 5608) [order 1] : % accelerometer quick calibration [int8(cmd.param5) == 4]
      (junction 5608) -> (junction 5609) : % _worker_thread.startTask(WorkerThread::Request::AccelCalibrationQuick); {answer_command(cmd, uint8(PX4_VEHICLE_COMMAND.VEHICLE_CMD_RESULT_ACCEPTED)); vehicle_status_flags_out_.condition_calibration_enabled = true;}
      (junction 5607) -> (junction 5610) [order 2]
      (junction 5609) -> (junction 5612)
      (junction 5610) -> (junction 5611) [order 1] : % airspeed calibration [int8(cmd.param6) == 1 || int8(cmd.param6) == 2]
      (junction 5611) -> (junction 5612) : % _worker_thread.startTask(WorkerThread::Request::AirspeedCalibration); {answer_command(cmd, uint8(PX4_VEHICLE_COMMAND.VEHICLE_CMD_RESULT_ACCEPTED)); vehicle_status_flags_out_.condition_calibration_enabled = true;}
      (junction 5610) -> (junction 5613) [order 2]
      (junction 5612) -> (junction 5615)
      (junction 5613) -> (junction 5614) [order 1] : % do esc calibration [int8(cmd.param7) == 1]
      (junction 5614) -> (junction 5615) : % function
      (junction 5613) -> (junction 5616) [order 2]
      (junction 5615) -> (junction 5618)
      (junction 5616) -> (junction 5617) [order 1] : % RC calibration ended - have we been in one worth confirming? [int8(cmd.param4) == 0]
      (junction 5617) -> (junction 5618) : % function
      (junction 5616) -> (junction 5619) [order 2]
      (junction 5618) -> (junction 5620)
      (junction 5620) -> (junction 5619)
      (junction 5619) -> (junction 5621)
    state FIXED_MAG_CAL_YAW [parallel]
      FIXED_MAG_CAL_YAW -> (junction 5683) : [hasChanged(cmd.timestamp) && ... cmd.command == PX4_VEHICLE_COMMAND.VEHICLE_CMD_FIXED_MAG_CAL_YAW]
      (junction 5683) -> (junction 5684) [order 1] : % reject if armed or shutting down % _worker_thread.isBusy() [vehicle_status_out_.arming_state == uint8(PX4_VEHICLE_STATUS.ARMING_STATE_ARMED) || ... vehicle_status_out_.arming_state == uint8(PX4_VEHICLE_STATUS.ARMING_STATE_SHUTDOWN)]
      (junction 5684) -> (junction 5685) : {answer_command(cmd, uint8(PX4_VEHICLE_COMMAND.VEHICLE_CMD_RESULT_TEMPORARILY_REJECTED));}
      (junction 5683) -> (junction 5686) [order 2] : {fixed_mag_cal_yaw(); answer_command(cmd, uint8(PX4_VEHICLE_COMMAND.VEHICLE_CMD_RESULT_ACCEPTED));}
      (junction 5685) -> (junction 5687)
      (junction 5687) -> (junction 5686)
      (junction 5686) -> (junction 5688)
    state PREFLIGHT_STORAGE [parallel]
      PREFLIGHT_STORAGE -> (junction 5698) : [hasChanged(cmd.timestamp) && ... cmd.command == PX4_VEHICLE_COMMAND.VEHICLE_CMD_PREFLIGHT_STORAGE]
      (junction 5698) -> (junction 5699) [order 1] : % _worker_thread.isBusy() [vehicle_status_out_.arming_state == uint8(PX4_VEHICLE_STATUS.ARMING_STATE_ARMED) || ... vehicle_status_out_.arming_state == uint8(PX4_VEHICLE_STATUS.ARMING_STATE_SHUTDOWN)]
      (junction 5699) -> (junction 5700) : % _worker_thread.startTask(WorkerThread::Request::ParamLoadDefault); {answer_command(cmd, uint8(PX4_VEHICLE_COMMAND.VEHICLE_CMD_RESULT_TEMPORARILY_REJECTED));}
      (junction 5698) -> (junction 5701) [order 2]
      (junction 5700) -> (junction 5703)
      (junction 5701) -> (junction 5702) [order 1] : [int8(cmd.param1) == 0]
      (junction 5702) -> (junction 5703) : % _worker_thread.startTask(WorkerThread::Request::ParamSaveDefault); {answer_command(cmd, uint8(PX4_VEHICLE_COMMAND.VEHICLE_CMD_RESULT_ACCEPTED));}
      (junction 5701) -> (junction 5704) [order 2]
      (junction 5703) -> (junction 5706)
      (junction 5704) -> (junction 5705) [order 1] : [int8(cmd.param1) == 1]
      (junction 5705) -> (junction 5706) : % answer_command(cmd, vehicle_command_s::VEHICLE_CMD_RESULT_ACCEPTED); {answer_command(cmd, uint8(PX4_VEHICLE_COMMAND.VEHICLE_CMD_RESULT_ACCEPTED));}
      (junction 5704) -> (junction 5707) [order 2]
      (junction 5706) -> (junction 5709)
      (junction 5707) -> (junction 5708) [order 1] : [int8(cmd.param1) == 2]
      (junction 5708) -> (junction 5709) : {answer_command(cmd, uint8(PX4_VEHICLE_COMMAND.VEHICLE_CMD_RESULT_ACCEPTED));}
      (junction 5707) -> (junction 5710) [order 2]
      (junction 5709) -> (junction 5711)
      (junction 5711) -> (junction 5710)
      (junction 5710) -> (junction 5712)
  state failure_detector_update [parallel]
    state updateAttitudeStatus [parallel]
      en,du:
      previous_status_ = status_;
      state disable_attitude_control
        en:
        status_ = bitand(status_, 0x00);
      state enable_attitude_control
        en,du:
        eulZYX = quat2eul(vehicle_attitude.q', 'ZYX');
        roll = eulZYX(3);
        pitch = eulZYX(2);
        max_roll = single(deg2rad(single(FD_FAIL_R)));
        max_pitch = single(deg2rad(single(FD_FAIL_P)));
        roll_status = (max_roll > 0.0) && (abs(roll) > max_roll);
        pitch_status = (max_pitch > 0.0) && (abs(pitch) > max_pitch);
        state roll [parallel]
          state roll_safe
            en:
            status_ = bitset(status_, FAILURE_ROLL, 0);
          state roll_failure
            en:
            status_ = bitset(status_, FAILURE_ROLL, 1);
          (default) -> roll_safe
          roll_safe -> roll_failure : [duration(roll_status, sec) > FD_FAIL_R_TTRI]
          roll_failure -> roll_safe : [~roll_status]
        state pitch [parallel]
          state pitch_safe
            en:
            status_ = bitset(status_, FAILURE_PITCH, 0);
          state pitch_failure
            en:
            status_ = bitset(status_, FAILURE_PITCH, 1);
          (default) -> pitch_safe
          pitch_safe -> pitch_failure : [duration(roll_status, sec) > FD_FAIL_P_TTRI]
          pitch_failure -> pitch_safe : [~pitch_status]
      (default) -> disable_attitude_control
      disable_attitude_control -> enable_attitude_control : [control_mode_out_.flag_control_attitude_enabled]
      enable_attitude_control -> disable_attitude_control : [~control_mode_out_.flag_control_attitude_enabled]
    state updateExternalAtsStatus [parallel]
      state none
      state run
        en,du:
        if hasChanged(pwm_input.timestamp)
        pulse_width = pwm_input.pulse_width;
        ats_trigger_status = (pulse_width > uint32(FD_EXT_ATS_TRIG)) && (pulse_width < 3000);
        end
        state ats_safe
          en:
          status_ = bitset(status_, FAILURE_EXT, 0);
        state ats_failure
          en:
          status_ = bitset(status_, FAILURE_EXT, 1);
        (default) -> ats_safe
        ats_safe -> ats_failure : [duration(ats_trigger_status, msec) > 100]
        ats_failure -> ats_safe : [~ats_trigger_status]
      (default) -> none
      none -> run : [FD_EXT_ATS_EN]
      run -> none : [~FD_EXT_ATS_EN]
    state esc_status_update [parallel]
      en,du:
      if hasChanged(esc_status.timestamp) && (vehicle_status_out_.arming_state == uint8(PX4_VEHICLE_STATUS.ARMING_STATE_ARMED))
      all_escs_armed = int8(bitshift(1, esc_status.esc_count) - 1);
      end
      state disable_esc_check
        en:
        % reset ESC bitfield
        status_ = bitand(status_, FAILURE_ARM_ESCS - 1);
      state enable_esc_check
        en:
        % set ESC bitfield
        status_ = bitor(status_, FAILURE_ARM_ESCS);
      (default) -> disable_esc_check
      disable_esc_check -> enable_esc_check : [FD_ESCS_EN && duration(all_escs_armed ~= esc_status.esc_armed_flags, msec) > 300]
      enable_esc_check -> disable_esc_check : [all_escs_armed == esc_status.esc_armed_flags]
    state failure_action [parallel]
      failure_action -> (junction 6531) : [status_ ~= previous_status_]
      (junction 6531) -> (junction 6532) : {vehicle_status_out_.failure_detector_status = status_; g_status_changed = true;}
      (junction 6532) -> (junction 6533) [order 1] : [actuator_armed_out_.armed]
      (junction 6533) -> (junction 6534) [order 1] : % 500ms is the PWM spoolup time. Within this timeframe controllers are not affecting actuator_outputs [bitand(vehicle_status_out_.failure_detector_status, FAILURE_ARM_ESCS) && ... uint64(getSimulationTime*1e+6) - vehicle_status_out_.armed_time < 500*1000]
      (junction 6534) -> (junction 6535) : % disarm(arm_disarm_reason_t::FAILURE_DETECTOR); {sprintf("mavlink_log_critical, ESCs did not respond to arm request")}
      (junction 6532) -> (junction 6544) [order 2]
      (junction 6533) -> (junction 6536) [order 2]
      (junction 6535) -> (junction 6540)
      (junction 6536) -> (junction 6537) [order 1] : [bitand(vehicle_status_out_.failure_detector_status, FAILURE_ROLL) || ... bitand(vehicle_status_out_.failure_detector_status, FAILURE_PITCH) || ... bitand(vehicle_status_out_.failure_detector_status, FAILURE_ALT) || ... bitand(vehicle_status_out_.failure_detector_status, FAILURE_EXT) ]
      (junction 6537) -> (junction 6538) : {is_second_after_takeoff = (uint64(getSimulationTime*1e+6) - vehicle_status_out_.takeoff_time) < (COM_LKDOWN_TKO* 1e+6);}
      (junction 6538) -> (junction 6539) [order 1] : [is_second_after_takeoff && ~lockdown_triggered_]
      (junction 6539) -> (junction 6540) : % This handles the case where something fails during the early takeoff phase {actuator_armed_out_.lockdown = true; lockdown_triggered_ = true; sprintf("mavlink_log_emergency, Critical failure detected: lockdown")}
      (junction 6538) -> (junction 6541) [order 2]
      (junction 6536) -> (junction 6545) [order 2]
      (junction 6540) -> (junction 6543)
      (junction 6541) -> (junction 6542) [order 1] : [~vehicle_status_flags_out_.circuit_breaker_flight_termination_disabled && ... ~flight_termination_triggered_ && ~lockdown_triggered_]
      (junction 6542) -> (junction 6543) : % set_tune_override(tune_control_s::TUNE_ID_PARACHUTE_RELEASE); {actuator_armed_out_.force_failsafe = true; flight_termination_triggered_ = true; sprintf("mavlink_log_emergency, Critical failure detected: terminate flight")}
      (junction 6541) -> (junction 6546) [order 2]
      (junction 6543) -> (junction 6547)
      (junction 6545) -> (junction 6544)
      (junction 6546) -> (junction 6545)
      (junction 6547) -> (junction 6546)
      (junction 6544) -> (junction 6548)
  state arming_state_transition [parallel]
    en,du:
    hil_enabled = (vehicle_status_out_.hil_state == PX4_VEHICLE_STATUS.HIL_STATE_ON);
    state init_precheck
      en:
    state standby_error [commented out]
      en:
    state standby
      % e.g. disarm
      state hil_enable [parallel]
        en:
        if (hil_enabled)
        g_status_changed = true;
        % enforce lockdown in HIL
        actuator_armed_out_.lockdown = true;
        vehicle_status_flags_out_.condition_system_sensors_initialized = true;
        % recover from a prearm fail
        if (vehicle_status_out_.arming_state == uint8(PX4_VEHICLE_STATUS.ARMING_STATE_STANDBY_ERROR))
        vehicle_status_out_.arming_state = uint8(PX4_VEHICLE_STATUS.ARMING_STATE_STANDBY);
        end
        % HIL can always go to standby
        % if (new_arming_state == vehicle_status_s::ARMING_STATE_STANDBY)
        % valid_transition = true;
        % end
        end
      state disarm_by_safety_button [parallel]
        en:
        if ~hil_enabled && vehicle_status_flags_out_.condition_system_sensors_initialized
        g_status_changed = true;
        actuator_armed_out_.armed = false;
        actuator_armed_out_.ready_to_arm = true;
        vehicle_status_out_.arming_state = uint8(PX4_VEHICLE_STATUS.ARMING_STATE_STANDBY);
        vehicle_status_out_.latest_disarming_reason = uint8(PX4_ARM_DISARM_REASON.SAFETY_BUTTON);
        vehicle_status_out_.armed_time = uint64(0);
        sprintf("mavlink_log_info, Disarmed by safety button");
        end
      state arm_state_trans_to_standby [parallel]
        en:
        % If arming_state in INIT state, try to proceed to STANDBY state
        if ~hil_enabled && ~vehicle_status_flags_out_.condition_calibration_enabled && ...
        vehicle_status_out_.arming_state == PX4_VEHICLE_STATUS.ARMING_STATE_INIT
        arm_state_in_init_tans_to_standby();
        end
    state armed
      en,du:
    state in_air_restore [commented out]
      en:
    state shutdown [commented out]
    init_precheck -> standby_error [commented out]
    (default) -> init_precheck
    standby_error -> init_precheck [commented out]
    standby -> standby_error [commented out]
    init_precheck -> standby : [EVT_DISARM || ... ~vehicle_status_flags_out_.condition_calibration_enabled]
    standby -> init_precheck [commented out] : % preflightcheck
    armed -> standby_error [commented out]
    standby -> armed : [EVT_ARM_RC_STICK]
    armed -> in_air_restore [commented out]
    armed -> standby : [EVT_AUTO_DISARM_LAND || ... EVT_AUTO_DISARM_PREFLIGHT || ... EVT_SAFETY_BUTTON || ... EVT_ARM_RC_STICK]
    in_air_restore -> armed [commented out]
    standby -> shutdown [commented out] : [ ]
  state set_navigation_state [parallel]
    % Check failsafe and main status and set navigation status for navigator accordingly
    % now set navigation state according to failsafe and main state
    note: 1、main_state_transition cmd => internal， function, or using state + event 2、set_nav_state() internal ==> status ==>publish, always 3、status ==> flag
    state prepare_params [parallel]
      en,du:
      nav_state_old = vehicle_status_out_.nav_state;
      data_link_loss_act_configured = NAV_DLL_ACT > uint8(PX4_LINK_LOSS_ACTIONS.DISABLED);
      rc_loss_act_configured = NAV_RCL_ACT > uint8(PX4_LINK_LOSS_ACTIONS.DISABLED);
      rc_lost = rc_loss_act_configured && vehicle_status_out_.rc_signal_lost;
      is_armed = (vehicle_status_out_.arming_state == PX4_VEHICLE_STATUS.ARMING_STATE_ARMED);
      old_failsafe = vehicle_status_out_.failsafe;
      vehicle_status_out_.failsafe = false;
    state rc_link_lost_act [parallel]
      rc_link_lost_act -> (junction 5943) : [old_failsafe]
      (junction 5943) -> (junction 5944) [order 1] : [NAV_RCL_ACT == uint8(PX4_LINK_LOSS_ACTIONS.TERMINATE) || ... NAV_DLL_ACT == uint8(PX4_LINK_LOSS_ACTIONS.TERMINATE)]
      (junction 5944) -> (junction 5945) : {actuator_armed_out_.force_failsafe = false;}
      (junction 5943) -> (junction 5946) [order 2]
      (junction 5945) -> (junction 5948)
      (junction 5946) -> (junction 5947) [order 1] : [NAV_RCL_ACT == uint8(PX4_LINK_LOSS_ACTIONS.TERMINATE) || ... NAV_DLL_ACT == uint8(PX4_LINK_LOSS_ACTIONS.TERMINATE)]
      (junction 5947) -> (junction 5948) : {actuator_armed_out_.lockdown = false;}
      (junction 5946) -> (junction 5949) [order 2]
      (junction 5948) -> (junction 5950)
      (junction 5950) -> (junction 5949)
      (junction 5949) -> (junction 5951)
    state offb_lost_act [parallel]
      offb_lost_act -> (junction 5964) : [old_failsafe]
      (junction 5964) -> (junction 5965) [order 1] : [COM_OBL_ACT == int8(PX4_OFFBOARD_LOSS_ACTIONS.TERMINATE) || ... COM_OBL_RC_ACT == int8(PX4_OFFBOARD_LOSS_RC_ACTIONS.TERMINATE) ]
      (junction 5965) -> (junction 5966) : {actuator_armed_out_.force_failsafe = false;}
      (junction 5964) -> (junction 5967) [order 2]
      (junction 5966) -> (junction 5969)
      (junction 5967) -> (junction 5968) [order 1] : [COM_OBL_ACT == int8(PX4_OFFBOARD_LOSS_ACTIONS.LOCKDOWN) || ... COM_OBL_RC_ACT == int8(PX4_OFFBOARD_LOSS_RC_ACTIONS.LOCKDOWN)]
      (junction 5968) -> (junction 5969) : {actuator_armed_out_.lockdown = false;}
      (junction 5967) -> (junction 5970) [order 2]
      (junction 5969) -> (junction 5971)
      (junction 5971) -> (junction 5970)
      (junction 5970) -> (junction 5972)
    state MAIN_STATE_ACRO [parallel]
      MAIN_STATE_ACRO -> (junction 5985) : [(internal_state_out_.main_state == PX4_COMMANDER_STATE.MAIN_STATE_ACRO) || ... (internal_state_out_.main_state == PX4_COMMANDER_STATE.MAIN_STATE_MANUAL) || ... (internal_state_out_.main_state == PX4_COMMANDER_STATE.MAIN_STATE_STAB) || ... (internal_state_out_.main_state == PX4_COMMANDER_STATE.MAIN_STATE_ALTCTL)]
      (junction 5985) -> (junction 5986) [order 1] : % require RC for all manual modes [rc_lost && is_armed]
      (junction 5986) -> (junction 5987) : {set_navigation_state.enable_failsafe("No manual control stick input"); set_navigation_state.set_link_loss_nav_state(NAV_RCL_ACT, COM_RCL_ACT_T);}
      (junction 5985) -> (junction 5988) [order 2]
      (junction 5987) -> (junction 5990)
      (junction 5988) -> (junction 5989) [order 1] : [internal_state_out_.main_state == PX4_COMMANDER_STATE.MAIN_STATE_ACRO]
      (junction 5989) -> (junction 5990) : {vehicle_status_out_.nav_state = uint8(PX4_VEHICLE_STATUS.NAVIGATION_STATE_ACRO);}
      (junction 5988) -> (junction 5991) [order 2]
      (junction 5990) -> (junction 5993)
      (junction 5991) -> (junction 5992) [order 1] : [internal_state_out_.main_state == PX4_COMMANDER_STATE.MAIN_STATE_MANUAL]
      (junction 5992) -> (junction 5993) : {vehicle_status_out_.nav_state = uint8(PX4_VEHICLE_STATUS.NAVIGATION_STATE_MANUAL);}
      (junction 5991) -> (junction 5994) [order 2]
      (junction 5993) -> (junction 5996)
      (junction 5994) -> (junction 5995) [order 1] : [internal_state_out_.main_state == PX4_COMMANDER_STATE.MAIN_STATE_STAB]
      (junction 5995) -> (junction 5996) : {vehicle_status_out_.nav_state = uint8(PX4_VEHICLE_STATUS.NAVIGATION_STATE_STAB);}
      (junction 5994) -> (junction 5997) [order 2]
      (junction 5996) -> (junction 5999)
      (junction 5997) -> (junction 5998) [order 1] : [internal_state_out_.main_state == PX4_COMMANDER_STATE.MAIN_STATE_ALTCTL]
      (junction 5998) -> (junction 5999) : {vehicle_status_out_.nav_state = uint8(PX4_VEHICLE_STATUS.NAVIGATION_STATE_ALTCTL);}
      (junction 5997) -> (junction 6000) [order 2] : {vehicle_status_out_.nav_state = uint8(PX4_VEHICLE_STATUS.NAVIGATION_STATE_MANUAL);}
      (junction 5999) -> (junction 6001)
      (junction 6001) -> (junction 6000)
      (junction 6000) -> (junction 6002)
    state MAIN_STATE_POSCTL [parallel]
      MAIN_STATE_POSCTL -> (junction 6028) : [internal_state_out_.main_state == PX4_COMMANDER_STATE.MAIN_STATE_ACRO]
      (junction 6028) -> (junction 6029) : {rc_fallback_allowed = (COM_POSCTL_NAVL ~= PX4_POSITION_NAV_LOSS_ACTIONS.LAND_TERMINATE) || ~is_armed;}
      (junction 6029) -> (junction 6030) [order 1] : [rc_lost && is_armed]
      (junction 6030) -> (junction 6031) : % As long as there is RC, we can fallback to ALTCTL, or STAB.  % A local position estimate is enough for POSCTL for multirotors, % this enables POSCTL using e.g. flow. % For fixedwing, a global position is needed.  {set_navigation_state.enable_failsafe("No manual control stick input"); set_navigation_state.set_link_loss_nav_state(NAV_RCL_ACT, COM_RCL_ACT_T);}
      (junction 6029) -> (junction 6032) [order 2]
      (junction 6031) -> (junction 6034)
      (junction 6032) -> (junction 6033) [order 1] : [set_navigation_state.check_invalid_pos_nav_state(rc_fallback_allowed, ... vehicle_status_out_.vehicle_type == PX4_VEHICLE_STATUS.VEHICLE_TYPE_FIXED_WING)]
      (junction 6033) -> (junction 6034) : % nothing to do - everything done in check_invalid_pos_nav_state
      (junction 6032) -> (junction 6035) [order 2] : {vehicle_status_out_.nav_state = uint8(PX4_VEHICLE_STATUS.NAVIGATION_STATE_POSCTL);}
      (junction 6034) -> (junction 6036)
      (junction 6036) -> (junction 6035)
      (junction 6035) -> (junction 6037)
    state MAIN_STATE_AUTO_MISSION [parallel]
      note: 进入failsafe的三种情况： engine failure vtol转换失败 data and link丢失
      MAIN_STATE_AUTO_MISSION -> (junction 6060) : [internal_state_out_.main_state == PX4_COMMANDER_STATE.MAIN_STATE_AUTO_MISSION]
      (junction 6061) -> (junction 6062) : % nothing to do - everything done in check_invalid_pos_nav_state
      (junction 6060) -> (junction 6061) [order 1] : [is_armed && set_navigation_state.check_invalid_pos_nav_state(false, true)]
      (junction 6060) -> (junction 6063) [order 2]
      (junction 6062) -> (junction 6065)
      (junction 6063) -> (junction 6064) [order 1] : [vehicle_status_out_.engine_failure]
      (junction 6064) -> (junction 6065) : {vehicle_status_out_.nav_state = uint8(PX4_VEHICLE_STATUS.NAVIGATION_STATE_AUTO_LANDENGFAIL);}
      (junction 6063) -> (junction 6066) [order 2]
      (junction 6065) -> (junction 6068)
      (junction 6066) -> (junction 6067) [order 1] : [vehicle_status_flags_out_.vtol_transition_failure]
      (junction 6067) -> (junction 6068) : {vehicle_status_out_.nav_state = uint8(PX4_VEHICLE_STATUS.NAVIGATION_STATE_AUTO_RTL);}
      (junction 6066) -> (junction 6069) [order 2]
      (junction 6068) -> (junction 6071)
      (junction 6069) -> (junction 6070) [order 1] : [vehicle_status_out_.mission_failure]
      (junction 6070) -> (junction 6071) : {vehicle_status_out_.nav_state = uint8(PX4_VEHICLE_STATUS.NAVIGATION_STATE_AUTO_RTL);}
      (junction 6069) -> (junction 6072) [order 2]
      (junction 6071) -> (junction 6074)
      (junction 6072) -> (junction 6073) [order 1] : [vehicle_status_out_.data_link_lost && ... data_link_loss_act_configured && is_armed && ~land_detector.landed]
      (junction 6073) -> (junction 6074) : % Data link lost, data link loss reaction configured -> do configured reaction {set_navigation_state.enable_failsafe("no datalink"); set_navigation_state.set_link_loss_nav_state(NAV_DLL_ACT, 0);}
      (junction 6072) -> (junction 6075) [order 2]
      (junction 6074) -> (junction 6077)
      (junction 6075) -> (junction 6076) [order 1] : [vehicle_status_out_.rc_signal_lost && rc_loss_act_configured && ... vehicle_status_flags_out_.rc_signal_found_once && is_armed && ~land_detector.landed]
      (junction 6076) -> (junction 6077) : % RC link lost, rc loss reaction configured, RC was used before -> RC loss reaction after delay % Safety pilot expects to be able to take over by RC in case anything unexpected happens {set_navigation_state.enable_failsafe("No manual control stick input"); set_navigation_state.set_link_loss_nav_state(NAV_RCL_ACT, COM_RCL_ACT_T);}
      (junction 6075) -> (junction 6078) [order 2]
      (junction 6077) -> (junction 6080)
      (junction 6078) -> (junction 6079) [order 1] : [vehicle_status_out_.rc_signal_lost && rc_loss_act_configured && ... vehicle_status_out_.data_link_lost && ... ~data_link_loss_act_configured && is_armed && ~land_detector.landed]
      (junction 6079) -> (junction 6080) : % All links lost, no data link loss reaction configured -> immediately do RC loss reaction % Lost all communication, by default it's considered unsafe to continue the mission % Note this case is reached after the previous one when flying mission completely without RC {set_navigation_state.enable_failsafe("no datalink"); set_navigation_state.set_link_loss_nav_state(NAV_RCL_ACT, 0);}
      (junction 6078) -> (junction 6081) [order 2]
      (junction 6080) -> (junction 6083)
      (junction 6081) -> (junction 6082) [order 1] : [vehicle_status_out_.rc_signal_lost && ~rc_loss_act_configured && ... vehicle_status_out_.data_link_lost && ~data_link_loss_act_configured && ... is_armed && ~land_detector.landed && mission_result.finished]
      (junction 6082) -> (junction 6083) : % All links lost, all link loss reactions disabled -> return after mission % Pilot disabled all reactions, finish mission but then return to avoid lost vehicle {set_navigation_state.enable_failsafe("no datalink"); set_navigation_state.set_link_loss_nav_state(int32(PX4_LINK_LOSS_ACTIONS.AUTO_RTL), 0);}
      (junction 6081) -> (junction 6084) [order 2]
      (junction 6083) -> (junction 6086)
      (junction 6084) -> (junction 6085) [order 1] : [~mission_result.stay_in_failsafe]
      (junction 6085) -> (junction 6086) : % normal mission operation if there's no need to stay in failsafe {vehicle_status_out_.nav_state = uint8(PX4_VEHICLE_STATUS.NAVIGATION_STATE_AUTO_MISSION);}
      (junction 6084) -> (junction 6087) [order 2]
      (junction 6086) -> (junction 6088)
      (junction 6088) -> (junction 6087)
      (junction 6087) -> (junction 6089)
    state MAIN_STATE_AUTO_LOITER [parallel]
      MAIN_STATE_AUTO_LOITER -> (junction 6131) : [internal_state_out_.main_state == PX4_COMMANDER_STATE.MAIN_STATE_AUTO_LOITER]
      (junction 6131) -> (junction 6132) [order 1] : % go into failsafe on a engine failure [vehicle_status_out_.engine_failure]
      (junction 6132) -> (junction 6133) : {vehicle_status_out_.nav_state = uint8(PX4_VEHICLE_STATUS.NAVIGATION_STATE_AUTO_LANDENGFAIL);}
      (junction 6131) -> (junction 6134) [order 2]
      (junction 6133) -> (junction 6136)
      (junction 6134) -> (junction 6135) [order 1] : [is_armed && set_navigation_state.check_invalid_pos_nav_state(false, true)]
      (junction 6135) -> (junction 6136) : % nothing to do - everything done in check_invalid_pos_nav_state
      (junction 6134) -> (junction 6137) [order 2]
      (junction 6136) -> (junction 6139)
      (junction 6137) -> (junction 6138) [order 1] : [vehicle_status_out_.data_link_lost && ... data_link_loss_act_configured && is_armed && ~land_detector.landed]
      (junction 6138) -> (junction 6139) : % also go into failsafe if just datalink is lost, and we're actually in air {set_navigation_state.enable_failsafe("no datalink"); set_navigation_state.set_link_loss_nav_state(NAV_DLL_ACT, 0);}
      (junction 6137) -> (junction 6140) [order 2]
      (junction 6139) -> (junction 6142)
      (junction 6140) -> (junction 6141) [order 1] : [rc_lost && ~rc_loss_act_configured && ... vehicle_status_out_.data_link_lost && ... ~data_link_loss_act_configured && is_armed]
      (junction 6141) -> (junction 6142) : % go into failsafe if RC is lost and datalink is lost and datalink loss is not set up {set_navigation_state.enable_failsafe("No manual control stick input"); set_navigation_state.set_link_loss_nav_state(NAV_RCL_ACT, 0);}
      (junction 6140) -> (junction 6143) [order 2]
      (junction 6142) -> (junction 6145)
      (junction 6143) -> (junction 6144) [order 1] : [vehicle_status_out_.rc_signal_lost]
      (junction 6144) -> (junction 6145) : % don't bother if RC is lost if datalink is connected  % this mode is ok, we don't need RC for LOITERing  {vehicle_status_out_.nav_state = uint8(PX4_VEHICLE_STATUS.NAVIGATION_STATE_AUTO_LOITER);}
      (junction 6143) -> (junction 6146) [order 2] : % everything is perfect {vehicle_status_out_.nav_state = uint8(PX4_VEHICLE_STATUS.NAVIGATION_STATE_AUTO_LOITER);}
      (junction 6145) -> (junction 6147)
      (junction 6147) -> (junction 6146)
      (junction 6146) -> (junction 6148)
    state MAIN_STATE_AUTO_RTL [parallel]
      MAIN_STATE_AUTO_RTL -> (junction 6173) : [internal_state_out_.main_state == PX4_COMMANDER_STATE.MAIN_STATE_AUTO_RTL]
      (junction 6173) -> (junction 6174) [order 1] : % require global position and home, also go into failsafe on an engine failure [vehicle_status_out_.engine_failure]
      (junction 6174) -> (junction 6175) : {vehicle_status_out_.nav_state = uint8(PX4_VEHICLE_STATUS.NAVIGATION_STATE_AUTO_LANDENGFAIL);}
      (junction 6173) -> (junction 6176) [order 2]
      (junction 6175) -> (junction 6178)
      (junction 6176) -> (junction 6177) [order 1] : [is_armed && set_navigation_state.check_invalid_pos_nav_state(false, true)]
      (junction 6177) -> (junction 6178) : % nothing to do - everything done in check_invalid_pos_nav_state
      (junction 6176) -> (junction 6179) [order 2] : {vehicle_status_out_.nav_state = uint8(PX4_VEHICLE_STATUS.NAVIGATION_STATE_AUTO_RTL);}
      (junction 6178) -> (junction 6180)
      (junction 6180) -> (junction 6179)
      (junction 6179) -> (junction 6181)
    state MAIN_STATE_AUTO_FOLLOW_TARGET [parallel]
      MAIN_STATE_AUTO_FOLLOW_TARGET -> (junction 6194) : [internal_state_out_.main_state == PX4_COMMANDER_STATE.MAIN_STATE_AUTO_FOLLOW_TARGET]
      (junction 6194) -> (junction 6195) [order 1] : % require global position and home [vehicle_status_out_.engine_failure]
      (junction 6195) -> (junction 6196) : {vehicle_status_out_.nav_state = uint8(PX4_VEHICLE_STATUS.NAVIGATION_STATE_AUTO_LANDENGFAIL);}
      (junction 6194) -> (junction 6197) [order 2]
      (junction 6196) -> (junction 6199)
      (junction 6197) -> (junction 6198) [order 1] : [is_armed && set_navigation_state.check_invalid_pos_nav_state(false, true)]
      (junction 6198) -> (junction 6199) : % nothing to do - everything done in check_invalid_pos_nav_state
      (junction 6197) -> (junction 6200) [order 2] : {vehicle_status_out_.nav_state = uint8(PX4_VEHICLE_STATUS.NAVIGATION_STATE_AUTO_FOLLOW_TARGET);}
      (junction 6199) -> (junction 6201)
      (junction 6201) -> (junction 6200)
      (junction 6200) -> (junction 6202)
    state MAIN_STATE_ORBIT [parallel]
      MAIN_STATE_ORBIT -> (junction 6215) : [internal_state_out_.main_state == PX4_COMMANDER_STATE.MAIN_STATE_ORBIT]
      (junction 6215) -> (junction 6216) [order 1] : % failsafe: on engine failure [vehicle_status_out_.engine_failure]
      (junction 6216) -> (junction 6217) : % failsafe: on engine failure % Orbit can only be started via vehicle_command (mavlink). Recovery from failsafe into orbit % is not possible and therefore the internal_state needs to be adjusted. {vehicle_status_out_.nav_state = uint8(PX4_VEHICLE_STATUS.NAVIGATION_STATE_AUTO_LANDENGFAIL); internal_state_out_.main_state = uint8(PX4_COMMANDER_STATE.MAIN_STATE_POSCTL);}
      (junction 6215) -> (junction 6218) [order 2]
      (junction 6217) -> (junction 6220)
      (junction 6218) -> (junction 6219) [order 1] : [is_armed && set_navigation_state.check_invalid_pos_nav_state(false, true)]
      (junction 6219) -> (junction 6220) : % failsafe: necessary position estimate lost; switching is done in check_invalid_pos_nav_state % Orbit can only be started via vehicle_command (mavlink). Consequently, recovery from failsafe into orbit % is not possible and therefore the internal_state needs to be adjusted. {internal_state_out_.main_state = uint8(PX4_COMMANDER_STATE.MAIN_STATE_POSCTL);}
      (junction 6218) -> (junction 6221) [order 2]
      (junction 6220) -> (junction 6223)
      (junction 6221) -> (junction 6222) [order 1] : [vehicle_status_out_.data_link_lost && ... data_link_loss_act_configured && ~land_detector.landed && is_armed]
      (junction 6222) -> (junction 6223) : % failsafe: just datalink is lost and we're in air % Orbit can only be started via vehicle_command (mavlink). Consequently, recovery from failsafe into orbit % is not possible and therefore the internal_state needs to be adjusted. {set_navigation_state.set_link_loss_nav_state(NAV_DLL_ACT, 0); set_navigation_state.enable_failsafe("no datalink"); internal_state_out_.main_state = uint8(PX4_COMMANDER_STATE.MAIN_STATE_POSCTL);}
      (junction 6221) -> (junction 6224) [order 2]
      (junction 6223) -> (junction 6226)
      (junction 6224) -> (junction 6225) [order 1] : [rc_lost && vehicle_status_out_.data_link_lost && ... ~data_link_loss_act_configured && is_armed]
      (junction 6225) -> (junction 6226) : % Orbit does not depend on RC but while armed & all links lost & when datalink loss is not set up, we failsafe % Orbit can only be started via vehicle_command (mavlink). Consequently, recovery from failsafe into orbit % is not possible and therefore the internal_state needs to be adjusted. {set_navigation_state.enable_failsafe("No manual control stick input"); set_navigation_state.set_link_loss_nav_state(NAV_RCL_ACT, 0); internal_state_out_.main_state = uint8(PX4_COMMANDER_STATE.MAIN_STATE_POSCTL);}
      (junction 6224) -> (junction 6227) [order 2] : % no failsafe, RC is not mandatory for orbit {vehicle_status_out_.nav_state = uint8(PX4_VEHICLE_STATUS.NAVIGATION_STATE_ORBIT);}
      (junction 6226) -> (junction 6228)
      (junction 6228) -> (junction 6227)
      (junction 6227) -> (junction 6229)
    state MAIN_STATE_AUTO_TAKEOFF [parallel]
      MAIN_STATE_AUTO_TAKEOFF -> (junction 6254) : [internal_state_out_.main_state == PX4_COMMANDER_STATE.MAIN_STATE_AUTO_TAKEOFF]
      (junction 6254) -> (junction 6255) [order 1] : % require local position [vehicle_status_out_.engine_failure]
      (junction 6255) -> (junction 6256) : {vehicle_status_out_.nav_state = uint8(PX4_VEHICLE_STATUS.NAVIGATION_STATE_AUTO_LANDENGFAIL);}
      (junction 6254) -> (junction 6257) [order 2]
      (junction 6256) -> (junction 6259)
      (junction 6257) -> (junction 6258) [order 1] : [is_armed && set_navigation_state.check_invalid_pos_nav_state(false, false)]
      (junction 6258) -> (junction 6259) : % nothing to do - everything done in check_invalid_pos_nav_state
      (junction 6257) -> (junction 6260) [order 2] : {vehicle_status_out_.nav_state = uint8(PX4_VEHICLE_STATUS.NAVIGATION_STATE_AUTO_TAKEOFF);}
      (junction 6259) -> (junction 6261)
      (junction 6261) -> (junction 6260)
      (junction 6260) -> (junction 6262)
    state MAIN_STATE_AUTO_LAND [parallel]
      MAIN_STATE_AUTO_LAND -> (junction 6275) : [internal_state_out_.main_state == PX4_COMMANDER_STATE.MAIN_STATE_AUTO_LAND]
      (junction 6275) -> (junction 6276) [order 1] : % require local position [vehicle_status_out_.engine_failure]
      (junction 6276) -> (junction 6277) : {vehicle_status_out_.nav_state = uint8(PX4_VEHICLE_STATUS.NAVIGATION_STATE_AUTO_LANDENGFAIL);}
      (junction 6275) -> (junction 6278) [order 2]
      (junction 6277) -> (junction 6280)
      (junction 6278) -> (junction 6279) [order 1] : [is_armed && set_navigation_state.check_invalid_pos_nav_state(false, false)]
      (junction 6279) -> (junction 6280) : % nothing to do - everything done in check_invalid_pos_nav_state
      (junction 6278) -> (junction 6281) [order 2] : {vehicle_status_out_.nav_state = uint8(PX4_VEHICLE_STATUS.NAVIGATION_STATE_AUTO_LAND);}
      (junction 6280) -> (junction 6282)
      (junction 6282) -> (junction 6281)
      (junction 6281) -> (junction 6283)
    state MAIN_STATE_AUTO_PRECLAND [parallel]
      MAIN_STATE_AUTO_PRECLAND -> (junction 6296) : [internal_state_out_.main_state == PX4_COMMANDER_STATE.MAIN_STATE_AUTO_PRECLAND]
      (junction 6296) -> (junction 6297) [order 1] : % must be rotary wing plus same requirements as normal landing [vehicle_status_out_.engine_failure]
      (junction 6297) -> (junction 6298) : {vehicle_status_out_.nav_state = uint8(PX4_VEHICLE_STATUS.NAVIGATION_STATE_AUTO_LANDENGFAIL);}
      (junction 6296) -> (junction 6299) [order 2]
      (junction 6298) -> (junction 6301)
      (junction 6299) -> (junction 6300) [order 1] : [is_armed && set_navigation_state.check_invalid_pos_nav_state(false, false)]
      (junction 6300) -> (junction 6301) : % nothing to do - everything done in check_invalid_pos_nav_state
      (junction 6299) -> (junction 6302) [order 2] : {vehicle_status_out_.nav_state = uint8(PX4_VEHICLE_STATUS.NAVIGATION_STATE_AUTO_PRECLAND);}
      (junction 6301) -> (junction 6303)
      (junction 6303) -> (junction 6302)
      (junction 6302) -> (junction 6304)
    state MAIN_STATE_OFFBOARD [parallel]
      MAIN_STATE_OFFBOARD -> (junction 6317) : [internal_state_out_.main_state == PX4_COMMANDER_STATE.MAIN_STATE_OFFBOARD]
      (junction 6317) -> (junction 6318) [order 1] : [vehicle_status_flags_out_.offboard_control_signal_lost]
      (junction 6318) -> (junction 6319) [order 1] : [vehicle_status_out_.rc_signal_lost]
      (junction 6319) -> (junction 6320) : % Offboard and RC are lost {set_navigation_state.enable_failsafe("no RC and no offboard"); set_navigation_state.set_offboard_loss_nav_state(COM_OBL_ACT);}
      (junction 6317) -> (junction 6321) [order 2] : {vehicle_status_out_.nav_state = uint8(PX4_VEHICLE_STATUS.NAVIGATION_STATE_OFFBOARD);}
      (junction 6318) -> (junction 6322) [order 2] : % Offboard is lost, RC is ok {set_navigation_state.enable_failsafe("no offboard"); set_navigation_state.set_offboard_loss_rc_nav_state(COM_OBL_RC_ACT);}
      (junction 6320) -> (junction 6323)
      (junction 6322) -> (junction 6321)
      (junction 6323) -> (junction 6322)
      (junction 6321) -> (junction 6324)
    state STATUS_FLAGS [parallel]
      STATUS_FLAGS -> (junction 6336)
      (junction 6336) -> (junction 6337) [order 1] : [vehicle_status_out_.nav_state ~= nav_state_old]
      (junction 6337) -> (junction 6338) : {nav_state_changed_ = true; vehicle_status_out_.nav_state_timestamp = uint64(getSimulationTime*1e+6);}
      (junction 6336) -> (junction 6339) [order 2] : {nav_state_changed_ = false;}
      (junction 6338) -> (junction 6340)
      (junction 6340) -> (junction 6339)
      (junction 6339) -> (junction 6341)
      (junction 6341) -> (junction 6342) [order 1] : [vehicle_status_out_.failsafe ~= failsafe_old]
      (junction 6342) -> (junction 6343) : {g_status_changed = true;}
      (junction 6343) -> (junction 6344) [order 1] : [vehicle_status_out_.failsafe]
      (junction 6344) -> (junction 6345) : {sprintf("mavlink_log_info, Failsafe mode activated")}
      (junction 6341) -> (junction 6348) [order 2]
      (junction 6343) -> (junction 6346) [order 2]
      (junction 6345) -> (junction 6347)
      (junction 6346) -> (junction 6347) : {sprintf("Failsafe mode deactivated")}
      (junction 6347) -> (junction 6349)
      (junction 6349) -> (junction 6348)
      (junction 6348) -> (junction 6350) : {failsafe_old = vehicle_status_out_.failsafe;}
  state publish_states [parallel]
    state update_control_mode [function]
      (default) -> (junction 7169)
      (junction 7169) -> (junction 7170) : % set vehicle_control_mode according to set_navigation_state {control_mode_out_.flag_armed = false; % actuator_armed_out_.armed; 后续修改，还没写入就使用 control_mode_out_.flag_external_manual_override_ok = (~vehicle_status_out_.is_vtol && ... vehicle_status_out_.vehicle_type == PX4_VEHICLE_STATUS.VEHICLE_TYPE_FIXED_WING);}
      (junction 7170) -> (junction 7171) [order 1] : [vehicle_status_out_.nav_state == PX4_VEHICLE_STATUS.NAVIGATION_STATE_MANUAL]
      (junction 7171) -> (junction 7172) : {control_mode_out_.flag_control_manual_enabled = true; control_mode_out_.flag_control_rates_enabled = stabilization_required(); control_mode_out_.flag_control_attitude_enabled = stabilization_required();}
      (junction 7170) -> (junction 7173) [order 2]
      (junction 7172) -> (junction 7175)
      (junction 7173) -> (junction 7174) [order 1] : [vehicle_status_out_.nav_state == PX4_VEHICLE_STATUS.NAVIGATION_STATE_STAB]
      (junction 7174) -> (junction 7175) : {control_mode_out_.flag_control_manual_enabled = true; control_mode_out_.flag_control_rates_enabled = true; control_mode_out_.flag_control_attitude_enabled = true;}
      (junction 7173) -> (junction 7176) [order 2]
      (junction 7175) -> (junction 7178)
      (junction 7176) -> (junction 7177) [order 1] : [vehicle_status_out_.nav_state == PX4_VEHICLE_STATUS.NAVIGATION_STATE_ALTCTL]
      (junction 7177) -> (junction 7178) : {control_mode_out_.flag_control_manual_enabled = true; control_mode_out_.flag_control_rates_enabled = true; control_mode_out_.flag_control_attitude_enabled = true; control_mode_out_.flag_control_altitude_enabled = true; control_mode_out_.flag_control_climb_rate_enabled = true;}
      (junction 7176) -> (junction 7179) [order 2]
      (junction 7178) -> (junction 7181)
      (junction 7179) -> (junction 7180) [order 1] : [vehicle_status_out_.nav_state == PX4_VEHICLE_STATUS.NAVIGATION_STATE_POSCTL]
      (junction 7180) -> (junction 7181) : {control_mode_out_.flag_control_manual_enabled = true; control_mode_out_.flag_control_rates_enabled = true; control_mode_out_.flag_control_attitude_enabled = true; control_mode_out_.flag_control_altitude_enabled = true; control_mode_out_.flag_control_climb_rate_enabled = true; control_mode_out_.flag_control_position_enabled = ~vehicle_status_out_.in_transition_mode; control_mode_out_.flag_control_velocity_enabled = ~vehicle_status_out_.in_transition_mode;}
      (junction 7179) -> (junction 7182) [order 2]
      (junction 7181) -> (junction 7184)
      (junction 7182) -> (junction 7183) [order 1] : [vehicle_status_out_.nav_state == PX4_VEHICLE_STATUS.NAVIGATION_STATE_AUTO_RTL]
      (junction 7183) -> (junction 7184) : % override is not ok for the RTL and recovery mode  {control_mode_out_.flag_external_manual_override_ok = false;}
      (junction 7182) -> (junction 7185) [order 2]
      (junction 7184) -> (junction 7187)
      (junction 7185) -> (junction 7186) [order 1] : [vehicle_status_out_.nav_state == PX4_VEHICLE_STATUS.NAVIGATION_STATE_AUTO_FOLLOW_TARGET || ... vehicle_status_out_.nav_state == PX4_VEHICLE_STATUS.NAVIGATION_STATE_AUTO_LAND || ... vehicle_status_out_.nav_state == PX4_VEHICLE_STATUS.NAVIGATION_STATE_AUTO_LANDENGFAIL || ... vehicle_status_out_.nav_state == PX4_VEHICLE_STATUS.NAVIGATION_STATE_AUTO_PRECLAND || ... vehicle_status_out_.nav_state == PX4_VEHICLE_STATUS.NAVIGATION_STATE_AUTO_MISSION || ... vehicle_status_out_.nav_state == PX4_VEHICLE_STATUS.NAVIGATION_STATE_AUTO_LOITER || ... vehicle_status_out_.nav_state == PX4_VEHICLE_STATUS.NAVIGATION_STATE_AUTO_TAKEOFF]
      (junction 7186) -> (junction 7187) : {control_mode_out_.flag_control_auto_enabled = true; control_mode_out_.flag_control_rates_enabled = true; control_mode_out_.flag_control_attitude_enabled = true; control_mode_out_.flag_control_altitude_enabled = true; control_mode_out_.flag_control_climb_rate_enabled = true; control_mode_out_.flag_control_position_enabled = ~vehicle_status_out_.in_transition_mode; control_mode_out_.flag_control_velocity_enabled = ~vehicle_status_out_.in_transition_mode;}
      (junction 7185) -> (junction 7188) [order 2]
      (junction 7187) -> (junction 7190)
      (junction 7188) -> (junction 7189) [order 1] : [vehicle_status_out_.nav_state == PX4_VEHICLE_STATUS.NAVIGATION_STATE_AUTO_LANDGPSFAIL]
      (junction 7189) -> (junction 7190) : {control_mode_out_.flag_control_rates_enabled = true; control_mode_out_.flag_control_attitude_enabled = true; control_mode_out_.flag_control_climb_rate_enabled = true;}
      (junction 7188) -> (junction 7191) [order 2]
      (junction 7190) -> (junction 7193)
      (junction 7191) -> (junction 7192) [order 1] : [vehicle_status_out_.nav_state == PX4_VEHICLE_STATUS.NAVIGATION_STATE_ACRO]
      (junction 7192) -> (junction 7193) : {control_mode_out_.flag_control_manual_enabled = true; control_mode_out_.flag_control_rates_enabled = true;}
      (junction 7191) -> (junction 7194) [order 2]
      (junction 7193) -> (junction 7196)
      (junction 7194) -> (junction 7195) [order 1] : [vehicle_status_out_.nav_state == PX4_VEHICLE_STATUS.NAVIGATION_STATE_DESCEND]
      (junction 7195) -> (junction 7196) : {control_mode_out_.flag_control_auto_enabled = false; control_mode_out_.flag_control_rates_enabled = true; control_mode_out_.flag_control_attitude_enabled = true; control_mode_out_.flag_control_climb_rate_enabled = true;}
      (junction 7194) -> (junction 7197) [order 2]
      (junction 7196) -> (junction 7199)
      (junction 7197) -> (junction 7198) [order 1] : [vehicle_status_out_.nav_state == PX4_VEHICLE_STATUS.NAVIGATION_STATE_TERMINATION]
      (junction 7198) -> (junction 7199) : % disable all controllers on termination {control_mode_out_.flag_control_termination_enabled = true;}
      (junction 7197) -> (junction 7200) [order 2]
      (junction 7199) -> (junction 7202)
      (junction 7200) -> (junction 7201) [order 1] : [vehicle_status_out_.nav_state == PX4_VEHICLE_STATUS.NAVIGATION_STATE_OFFBOARD]
      (junction 7201) -> (junction 7202) : {set_offboard_flags();}
      (junction 7200) -> (junction 7203) [order 2]
      (junction 7202) -> (junction 7205)
      (junction 7203) -> (junction 7204) [order 1] : [vehicle_status_out_.nav_state == PX4_VEHICLE_STATUS.NAVIGATION_STATE_ORBIT]
      (junction 7204) -> (junction 7205) : {control_mode_out_.flag_control_manual_enabled = false; control_mode_out_.flag_control_auto_enabled = false; control_mode_out_.flag_control_rates_enabled = true; control_mode_out_.flag_control_attitude_enabled = true; control_mode_out_.flag_control_altitude_enabled = true; control_mode_out_.flag_control_climb_rate_enabled = true; control_mode_out_.flag_control_position_enabled = ~vehicle_status_out_.in_transition_mode; control_mode_out_.flag_control_velocity_enabled = ~vehicle_status_out_.in_transition_mode;}
      (junction 7203) -> (junction 7206) [order 2]
      (junction 7205) -> (junction 7207)
      (junction 7207) -> (junction 7206)
      (junction 7206) -> (junction 7208) : {control_mode_out_.timestamp = uint64(getSimulationTime*1e+6); control_mode_out_.flag_multicopter_position_control_enabled = ... (vehicle_status_out_.vehicle_type == PX4_VEHICLE_STATUS.VEHICLE_TYPE_ROTARY_WING) && ... (control_mode_out_.flag_control_altitude_enabled || ... control_mode_out_.flag_control_climb_rate_enabled || ... control_mode_out_.flag_control_position_enabled || ... control_mode_out_.flag_control_velocity_enabled || ... control_mode_out_.flag_control_acceleration_enabled);}
    publish_states -> (junction 6577) : % publish states (armed, control_mode, vehicle_status, commander_state, vehicle_status_flags) at 2 Hz or immediately when changed [(uint64(getSimulationTime*1e+6) - vehicle_status_out_.timestamp >= 50e+3) || ... g_status_changed || nav_state_changed_]
    (junction 6577) -> (junction 6579) : {update_control_mode();}
    (junction 6580) -> (junction 6578) : % skip prearmed state {actuator_armed_out_.prearmed = false;}
    (junction 6579) -> (junction 6580) [order 1] : [COM_PREARM_MODE == uint8(PX4_PREARMED_MODE.DISABLED)]
    (junction 6578) -> (junction 6583)
    (junction 6579) -> (junction 6581) [order 2]
    (junction 6581) -> (junction 6582) [order 1] : [COM_PREARM_MODE == uint8(PX4_PREARMED_MODE.SAFETY_BUTTON)]
    (junction 6582) -> (junction 6583) : % safety is not present, go into prearmed % * (all output drivers should be started / unlocked last in the boot process % * when the rest of the system is fully initialized) {actuator_armed_out_.prearmed = (uint64(getSimulationTime*1e+6) - boot_timestamp_) > 5*1e+6;}
    (junction 6581) -> (junction 6584) [order 2]
    (junction 6583) -> (junction 6587)
    (junction 6584) -> (junction 6585) [order 1] : [COM_PREARM_MODE == uint8(PX4_PREARMED_MODE.ALWAYS)]
    (junction 6585) -> (junction 6586) [order 1] : [safety_switch.safety_switch_available]
    (junction 6586) -> (junction 6587) : % safety switch is present, go into prearmed if safety is off  {actuator_armed_out_.prearmed = safety_switch.safety_off;}
    (junction 6584) -> (junction 6591) [order 2] : {actuator_armed_out_.prearmed = false;}
    (junction 6585) -> (junction 6589) [order 2]
    (junction 6587) -> (junction 6588)
    (junction 6589) -> (junction 6588) : % safety switch is not present, do not go into prearmed  {actuator_armed_out_.prearmed = false;}
    (junction 6588) -> (junction 6590)
    (junction 6590) -> (junction 6591)
    (junction 6591) -> (junction 6592) : % _commander_state_pub.publish(_internal_state); % _armed_pub.publish(_armed); % publish internal state for logging purposes  {actuator_armed_out_.timestamp = uint64(getSimulationTime*1e+6); internal_state_out_.timestamp = uint64(getSimulationTime*1e+6); evaluate_prearm_status();}
  state play_tunes [parallel]
    state arming_battery_tune [parallel]
      arming_battery_tune -> (junction 6713)
      (junction 6714) -> (junction 6715) : % play tune when armed  % set_tune(tune_control_s::TUNE_ID_ARMING_WARNING); {arm_tune_played_ = true;}
      (junction 6713) -> (junction 6714) [order 1] : [arm_tune_played_ && actuator_armed_out_.armed && ... (safety_switch.safety_switch_available || (safety_switch.safety_switch_available && safety_switch.safety_off))]
      (junction 6713) -> (junction 6716) [order 2]
      (junction 6715) -> (junction 6718)
      (junction 6716) -> (junction 6717) [order 1] : [~vehicle_status_flags_out_.usb_connected && ... (vehicle_status_out_.hil_state ~= PX4_VEHICLE_STATUS.HIL_STATE_ON) && ... (battery_warning_ == PX4_BATTERY_STATUS.BATTERY_WARNING_CRITICAL) ]
      (junction 6717) -> (junction 6718) : % play tune on battery critical  % set_tune(tune_control_s::TUNE_ID_BATTERY_WARNING_FAST);
      (junction 6716) -> (junction 6719) [order 2]
      (junction 6718) -> (junction 6721)
      (junction 6719) -> (junction 6720) [order 1] : [vehicle_status_out_.failsafe]
      (junction 6720) -> (junction 6721) : % tune_failsafe(true);
      (junction 6719) -> (junction 6722) [order 2] : % set_tune(tune_control_s::TUNE_ID_STOP);
      (junction 6721) -> (junction 6724)
      (junction 6723) -> (junction 6722)
      (junction 6724) -> (junction 6723)
      (junction 6722) -> (junction 6725)
    state reset_arm_tune [parallel]
      reset_arm_tune -> (junction 6743) : % reset arm_tune_played_ when disarmed  [~actuator_armed_out_.armed || ... (safety_switch.safety_switch_available && ~safety_switch.safety_off)]
      (junction 6743) -> (junction 6744) [order 1] : % Notify the user that it is safe to approach the vehicle [arm_tune_played_]
      (junction 6744) -> (junction 6745) : % tune_neutral(true);
      (junction 6743) -> (junction 6746) [order 2] : {arm_tune_played_ = false;}
      (junction 6745) -> (junction 6747)
      (junction 6747) -> (junction 6746)
      (junction 6746) -> (junction 6748)
    state sensor_failure_tune [parallel]
      sensor_failure_tune -> (junction 6759) : % play sensor failure tunes if we already waited for hotplug sensors to come up and failed  {sensor_fail_tune_played = false; vehicle_status_flags_out_.condition_system_hotplug_timeout = (uint64(getSimulationTime*1e+6) - boot_timestamp_ > HOTPLUG_SENS_TIMEOUT);}
      (junction 6759) -> (junction 6760) [order 1] : [~sensor_fail_tune_played && (~vehicle_status_flags_out_.condition_system_sensors_initialized && ... vehicle_status_flags_out_.condition_system_hotplug_timeout)]
      (junction 6760) -> (junction 6761) : % set_tune_override(tune_control_s::TUNE_ID_GPS_WARNING); {sensor_fail_tune_played = true; g_status_changed = true;}
      (junction 6759) -> (junction 6762) [order 2]
      (junction 6761) -> (junction 6763)
      (junction 6763) -> (junction 6762)
      (junction 6762) -> (junction 6764)
  state arm_auth_update [parallel]
  data: current_status function_input; ret function_output; current_status function_input; ret function_output; current_status function_input; ret function_output; is_rotary local boolean =false; is_fixed local boolean =false; is_ground local boolean =false; instance function_input; optional_mag function_input; is_report_mag_fail function_input; ret function_output; ret function_output; report_status function_input; report_mag_fail local boolean; ret function_output; instance function_input; optional_accel function_input; is_report_accel_fail function_input; report_accel_fail local boolean; ret function_output; instance function_input; optional_gyro function_input; is_report_gyro_fail function_input; report_gyro_fail local boolean; ret function_output; instance function_input; optional_baro function_input; is_report_baro_fail function_input; report_baro_fail local boolean; ret function_output; report_status function_input; optional_aspd function_input; report_failures function_input; prearm function_input; max_aspd_check_en function_input; arming_max_aspd_allowed function_input; ret function_output; airspeed_mode local int32 =int32(0); airspeed_trim local single =single(0); arming_max_airspeed_allowed local single =single(0); optional local boolean =false; is_report_rc_fail function_input; ret function_output; isVTOL function_input; ret function_output; report_power_fail function_input; prearm function_input; ret function_output; report_failure_fail function_input; ret function_output; report_ekf_fail function_input; report_bias_fail function_input; ret function_output; ekf_healthy local boolean =false; time_since_boot local uint64 =uint64(0); report_manual_fail function_input; ret function_output; ret function_output; report_cpu_fail function_input; i local uint8 =uint8(0); report_failures_ local boolean =false; report_fail local boolean =false; required local boolean =false; prearm_ local boolean =false; preflight_check_res_ local boolean =false; current_status function_input; ret function_output; current_status function_input; ret function_output; current_status function_input; ret function_output; CBRK_BUZZER_KEY constant single =782097; CBRK_SUPPLY_CHK_KEY constant single =894281; CBRK_RATE_CTRL_KEY constant single =140253; CBRK_IO_SAFETY_KEY constant single =22027; CBRK_AIRSPD_CHK_KEY constant single =162128; CBRK_FLIGHTTERM_KEY constant single =121212; CBRK_ENGINEFAIL_KEY constant single =284953; CBRK_USB_CHK_KEY constant single =197848; CBRK_VELPOSERR_KEY constant single =201607; CBRK_VTOLARMING_KEY constant single =159753; was_landed local boolean =true; INAIR_RESTART_HOLDOFF_INTERVAL constant uint64 =uint64(500); ref_pos local Bus: px4_map_projection_reference; home_lat local double; home_lon local double; home_alt local single; safety_disarm_allowed local boolean =false; new_vehicle_type local uint8 =uint8(0); should_soft_stop local boolean =false; last_esc_updated function_output; last_esc_status_updated local uint64 =uint64(0); nav_test_failed_ local boolean =false; nav_test_passed_ local boolean =false; batt_warn function_output; batt_warn_inc_while_armed function_output; battery_warning local uint8 =uint8(0); battery_warning_level_increased_while_armed local boolean =false; use_buzzer function_input; use_buzzer function_input; use_buzzer function_input; last_manual_control_setpoint local Bus: px4_manual_control_setpoint; rc_available local boolean =false; rc_allowed local boolean =false; rc_signal_lost_timestamp local uint64 =uint64(0); last_manual_control_switches_arm_switch local uint8 =uint8(0); last_change_disarm_time local uint64 =uint64(0); stick_disarm_hysteresis_state local boolean =false; last_stick_disarm_hysteresis_state local boolean =false; last_stick_arm_hysteresis_state local boolean =false; stick_arm_hysteresis_state local boolean =false; last_change_arm_time local uint64 =uint64(0); was_armed local boolean =false; timestamp_engine_healthy local uint64 =uint64(0); batteries local Bus: px4_battery_status; battery_current_ local single =single(0); base_mode local uint8 =uint8(0); custom_main_mode local uint8 =uint8(0); custom_sub_mode local uint8 =uint8(0); new_main_state local uint8 =uint8(0); param1_arm local single; cmd_arms local boolean; force local boolean; cmd_from_io local boolean; home_lat function_input; home_lon function_input; home_alt function_input; use_current local boolean; lat local double; lon local double; alt local single; throttle_type local int8; motor_count local int8; param1 local int8; heading_radians local single; cmd_result_ local uint8 =uint8(0); pulse_width local uint32 =uint32(0); ats_trigger_status local boolean =false; all_escs_armed local int8 =int8(0); is_second_after_takeoff local boolean =false; status_ local uint8 =uint8(0); eulZYX local single; roll local single; pitch local single; pitch_status local boolean =false; roll_status local boolean =false; max_roll local single; max_pitch local single; previous_status_ local uint8 =uint8(0); subsystem_type function_input; healthy function_input; status function_input; subsystem_type function_input; present function_input; enabled function_input; ok function_input; status function_input; data_valid function_input; data_accuracy function_input; required_accuracy function_input; data_timestamp_us function_input; last_fail_time_us function_input; probation_time_us function_input; was_valid function_input; ret function_output; hil_enabled local boolean =false; rc_fallback_allowed local boolean =false; reason function_input; link_loss_act function_input; ll_delay function_input; fallback_required function_output; use_rc function_input; using_global_pos function_input; offboard_loss_act function_input; offboard_loss_rc_act function_input; nav_state_old local uint8 =uint8(0); data_link_loss_act_configured local boolean =false; rc_loss_act_configured local boolean =false; rc_lost local boolean =false; is_armed local boolean =false; old_failsafe local boolean =false; failsafe_old local boolean =false; ret function_output; ret function_output boolean; home_pos function_input; lat function_input; lon function_input; alt function_input; home_pos function_input; local_pos function_input; gpos function_input Bus: px4_vehicle_global_position; ret function_output boolean; cmd_in function_input; result function_input; ret function_output; HOTPLUG_SENS_TIMEOUT constant uint64 =uint64(8*1e+6); sensor_fail_tune_played local boolean =false; arm_tune_played_ local boolean =false; ret function_output; new_main_state function_input; boot_timestamp_ local uint64 =uint64(0); last_lpos_fail_time_us_ local uint64 =uint64(0); last_gpos_fail_time_us_ local uint64 =uint64(0); last_lvel_fail_time_us_ local uint64 =uint64(0); vehicle_status_out_ output Bus: px4_vehicle_status; led_control_out_ output Bus: px4_led_control; tune_durations_ local uint32; CBRK_SUPPLY_CHK parameter; MAV_TYPE parameter; CBRK_USB_CHK parameter; CBRK_AIRSPD_CHK parameter; CBRK_ENGINEFAIL parameter; CBRK_FLIGHTTERM parameter; CBRK_VELPOSERR parameter; CBRK_VTOLARMING parameter; param_init_forced_ local boolean =true; VEHICLE_TYPE_FIXED_WING constant uint8 =uint8(1); VEHICLE_TYPE_QUADROTOR constant uint8 =uint8(2); VEHICLE_TYPE_COAXIAL constant uint8 =uint8(3); VEHICLE_TYPE_HELICOPTER constant uint8 =uint8(4); VEHICLE_TYPE_GROUND_ROVER constant uint8 =uint8(10); VEHICLE_TYPE_HEXAROTOR constant uint8 =uint8(13); VEHICLE_TYPE_OCTOROTOR constant uint8 =uint8(14); VEHICLE_TYPE_TRICOPTER constant uint8 =uint8(15); VEHICLE_TYPE_VTOL_DUOROTOR constant uint8 =uint8(19); VEHICLE_TYPE_VTOL_QUADROTOR constant uint8 =uint8(20); VEHICLE_TYPE_VTOL_TILTROTOR constant uint8 =uint8(21); VEHICLE_TYPE_VTOL_RESERVED2 constant uint8 =uint8(22); VEHICLE_TYPE_VTOL_RESERVED3 constant uint8 =uint8(23); VEHICLE_TYPE_VTOL_RESERVED4 constant uint8 =uint8(24); VEHICLE_TYPE_VTOL_RESERVED5 constant uint8 =uint8(25); MAV_SYS_ID parameter; COM_ARM_AUTH_TO parameter; param_com_arm_auth_timout_ local uint64 =uint64(0); COM_ARM_AUTH_MET parameter; COM_ARM_AUTH_ID parameter; params_update input Bus: px4_parameter_update; actuator_armed input Bus: px4_actuator_armed; vtol_status input Bus: px4_vtol_vehicle_status; g_status_changed local boolean =true; MAV_COMP_ID parameter; vehicle_status_flags_out_ output Bus: px4_vehicle_status_flags; COM_OBS_AVOID parameter; COM_RC_IN_MODE parameter; arm_requirements_ local px4_arm_requqirements; COM_ARM_AUTH_REQ parameter; COM_ARM_CHK_ESCS parameter; COM_ARM_MIS_REQ parameter; GF_ACTION parameter; flight_mode_slots_ local int32; COM_ARM_WO_GPS parameter; MC_AIRMODE parameter; RC_MAP_ARM_SW parameter; COM_FLTMODE1 parameter; COM_FLTMODE2 parameter; COM_FLTMODE3 parameter; COM_FLTMODE4 parameter; COM_FLTMODE5 parameter; COM_FLTMODE6 parameter; system_power input Bus: px4_system_power; land_detector input Bus: px4_vehicle_land_detected; COM_POS_FS_PROB parameter; gpos_probation_time_us_ local uint64 =uint64(0); lpos_probation_time_us_ local uint64 =uint64(0); lvel_probation_time_us_ local uint64 =uint64(0); home_position input Bus: px4_home_position; should_set_home_on_takeoff_ local boolean =true; COM_HOME_IN_AIR parameter; home_position_out_ output Bus: px4_home_position; local_position input Bus: px4_vehicle_local_position; global_position input Bus: px4_vehicle_global_position; COM_HOME_H_T parameter; COM_HOME_V_T parameter; safety_switch input Bus: px4_safety; SUBSYSTEM_TYPE_GYRO constant uint32 =bitshift(1,0); SUBSYSTEM_TYPE_ACC constant uint32 =bitshift(1,1); SUBSYSTEM_TYPE_MAG constant uint32 =bitshift(1,2); SUBSYSTEM_TYPE_ABSPRESSURE constant uint32 =bitshift(1,3); SUBSYSTEM_TYPE_DIFFPRESSURE constant uint32 =bitshift(1,4); SUBSYSTEM_TYPE_GPS constant uint32 =bitshift(1,5); SUBSYSTEM_TYPE_OPTICALFLOW constant uint32 =bitshift(1,6); SUBSYSTEM_TYPE_CVPOSITION constant uint32 =bitshift(1,7); SUBSYSTEM_TYPE_LASERPOSITION constant uint32 =bitshift(1,8); SUBSYSTEM_TYPE_EXTERNALGROUNDTRUTH constant uint32 =bitshift(1,9); SUBSYSTEM_TYPE_ANGULARRATECONTROL constant uint32 =bitshift(1,10); SUBSYSTEM_TYPE_ATTITUDESTABILIZATION constant uint32 =bitshift(1,11); SUBSYSTEM_TYPE_YAWPOSITION constant uint32 =bitshift(1,12); SUBSYSTEM_TYPE_ALTITUDECONTROL constant uint32 =bitshift(1,13); SUBSYSTEM_TYPE_POSITIONCONTROL constant uint32 =bitshift(1,14); SUBSYSTEM_TYPE_MOTORCONTROL constant uint32 =bitshift(1,15); SUBSYSTEM_TYPE_RCRECEIVER constant uint32 =bitshift(1,16); SUBSYSTEM_TYPE_GYRO2 constant uint32 =bitshift(1,17); SUBSYSTEM_TYPE_ACC2 constant uint32 =bitshift(1,18); SUBSYSTEM_TYPE_MAG2 constant uint32 =bitshift(1,19); SUBSYSTEM_TYPE_GEOFENCE constant uint32 =bitshift(1,20); SUBSYSTEM_TYPE_AHRS constant uint32 =bitshift(1,21); SUBSYSTEM_TYPE_TERRAIN constant uint32 =bitshift(1,22); SUBSYSTEM_TYPE_REVERSEMOTOR constant uint32 =bitshift(1,23); SUBSYSTEM_TYPE_LOGGING constant uint32 =bitshift(1,24); SUBSYSTEM_TYPE_SENSORBATTERY constant uint32 =bitshift(1,25); SUBSYSTEM_TYPE_SENSORPROXIMITY constant uint32 =bitshift(1,26); SUBSYSTEM_TYPE_SATCOM constant uint32 =bitshift(1,27); SUBSYSTEM_TYPE_PREARM_CHECK constant uint32 =bitshift(1,28); SUBSYSTEM_TYPE_OBSTACLE_AVOIDANCE constant uint32 =bitshift(1,29); actuator_armed_out_ output Bus: px4_actuator_armed; status_flags input Bus: px4_vehicle_status_flags; land_detector_ local Bus: px4_vehicle_land_detected; vtol_status_ local Bus: px4_vtol_vehicle_status; COM_DISARM_LAND parameter; COM_DISARM_PRFLT parameter; COM_KILL_DISARM parameter; battery_status input Bus: px4_battery_status; battery_status_out_ output Bus: px4_battery_status; rtl_flight_time input Bus: px4_rtl_flight_time; BAT_CRIT_THR parameter; BAT_LOW_THR parameter; COM_LOW_BAT_ACT parameter; BATTERY_FAILSAFE_WARNING constant uint8 =uint8(0); BATTERY_FAILSAFE_RETURN constant uint8 =uint8(1); BATTERY_FAILSAFE_LAND constant uint8 =uint8(2); BATTERY_FAILSAFE_RETURN_OR_LAND constant uint8 =uint8(3); internal_state_out_ output Bus: px4_commander_state; TRANSITION_DENIED constant int8 =int8(-1); TRANSITION_NOT_CHANGED constant int8 =int8(0); TRANSITION_CHANGED constant int8 =int8(1); SYS_HAS_MAG parameter; mission_result input Bus: px4_mission_result; COM_TAKEOFF_ACT parameter; actuator_controls input Bus: px4_actuator_controls; COM_EF_THROT parameter; COM_EF_C2T parameter; COM_EF_TIME parameter; cmd input Bus: px4_vehicle_command; VEHICLE_MODE_FLAG_CUSTOM_MODE_ENABLED constant uint8 =uint8(1); VEHICLE_MODE_FLAG_TEST_ENABLED constant uint8 =int8(2); VEHICLE_MODE_FLAG_AUTO_ENABLED constant uint8 =int8(4); VEHICLE_MODE_FLAG_GUIDED_ENABLED constant uint8 =int8(8); VEHICLE_MODE_FLAG_STABILIZE_ENABLED constant uint8 =int8(16); VEHICLE_MODE_FLAG_HIL_ENABLED constant uint8 =int8(32); VEHICLE_MODE_FLAG_MANUAL_INPUT_ENABLED constant uint8 =int8(64); VEHICLE_MODE_FLAG_SAFETY_ARMED constant uint8 =int8(128); VEHICLE_MODE_FLAG_ENUM_END constant uint8 =int8(129); POSVEL_PROBATION_MIN constant uint64 =int64(1e+6); COM_POS_FS_EPH parameter; COM_POS_FS_DELAY parameter; COM_POS_FS_GAIN parameter; lockdown_triggered_ local boolean =false; flight_termination_triggered_ local boolean =false; high_latency_datalink_heartbeat_ local uint64 =uint64(0); COM_MOT_TEST_EN parameter; test_motor_out_ output Bus: px4_test_motor; command_ack_out_ output Bus: px4_vehicle_command_ack; control_mode_out_ output Bus: px4_vehicle_control_mode; FAILURE_NONE constant uint8 =uint8(0); FAILURE_ROLL constant uint8 =uint8(1); FAILURE_PITCH constant uint8 =uint8(2); FAILURE_ALT constant uint8 =uint8(4); FAILURE_EXT constant uint8 =uint8(8); FAILURE_ARM_ESCS constant uint8 =uint8(16); vehicle_attitude input Bus: px4_vehicle_attitude; FD_FAIL_R parameter; FD_FAIL_P parameter; FD_FAIL_R_TTRI parameter; FD_FAIL_P_TTRI parameter; FD_EXT_ATS_EN parameter; pwm_input input Bus: px4_pwm_input; FD_EXT_ATS_TRIG parameter; FD_ESCS_EN parameter; esc_status input Bus: px4_esc_status; COM_LKDOWN_TKO parameter; last_disarmed_timestamp_ local uint64 =uint64(0); have_taken_off_since_arming_ local boolean =false; NAV_DLL_ACT parameter; NAV_RCL_ACT parameter; COM_OBL_RC_ACT parameter; COM_OBL_ACT parameter; COM_RCL_ACT_T parameter; COM_POSCTL_NAVL parameter; nav_state_changed_ local boolean =false; offboard_control_mode input Bus: px4_offboard_control_mode; COM_PREARM_MODE parameter; battery_warning_ local boolean =false; sensor_mag input Bus: px4_sensor_mag; sensor_accel input Bus: px4_sensor_accel; sensor_gyro input Bus: px4_sensor_gyro; sensor_baro input Bus: px4_sensor_baro; max_mandatory_gyro_count constant uint8 =uint8(1); max_optional_gyro_count constant uint8 =uint8(4); max_mandatory_accel_count constant uint8 =uint8(1); max_optional_accel_count constant uint8 =uint8(4); max_mandatory_mag_count constant uint8 =uint8(1); max_optional_mag_count constant uint8 =uint8(4); max_mandatory_baro_count constant uint8 =uint8(1); max_optional_baro_count constant uint8 =uint8(4); COM_ARM_MAG_ANG parameter; sensors input Bus: px4_sensor_preflight_mag; SYS_HAS_BARO parameter; COM_ARM_IMU_ACC parameter; COM_ARM_IMU_GYR parameter; sensors_status_imu input Bus: px4_sensors_status_imu; FW_ARSP_MODE parameter; COM_ARM_ARSP_EN parameter; FW_AIRSPD_TRIM parameter; airspeed_validated input Bus: px4_airspeed_validated; COM_POWER_COUNT parameter; manual_control_switches input Bus: px4_manual_control_switches; estimator_sensor_bias input Bus: px4_estimator_sensor_bias; estimator_selector_status input Bus: px4_estimator_selector_status; estimator_status input Bus: px4_estimator_status; cpuload input Bus: px4_cpuload; COM_CPU_MAX parameter; RC_MAP_TRANS_SW parameter; RC_INPUT_MAX_DEADZONE_US constant int16 =uint64(500); RC1_MIN parameter; RC2_MIN parameter; RC3_MIN parameter; RC4_MIN parameter; RC5_MIN parameter; RC6_MIN parameter; RC7_MIN parameter; RC8_MIN parameter; RC9_MIN parameter; RC10_MIN parameter; RC11_MIN parameter; RC12_MIN parameter; RC13_MIN parameter; RC14_MIN parameter; RC15_MIN parameter; RC16_MIN parameter; RC17_MIN parameter; RC18_MIN parameter; RC1_TRIM parameter; RC2_TRIM parameter; RC3_TRIM parameter; RC4_TRIM parameter; RC5_TRIM parameter; RC6_TRIM parameter; RC7_TRIM parameter; RC8_TRIM parameter; RC9_TRIM parameter; RC10_TRIM parameter; RC11_TRIM parameter; RC12_TRIM parameter; RC13_TRIM parameter; RC14_TRIM parameter; RC15_TRIM parameter; RC16_TRIM parameter; RC17_TRIM parameter; RC18_TRIM parameter; RC1_MAX parameter; RC2_MAX parameter; RC3_MAX parameter; RC4_MAX parameter; RC5_MAX parameter; RC6_MAX parameter; RC7_MAX parameter; RC8_MAX parameter; RC9_MAX parameter; RC10_MAX parameter; RC11_MAX parameter; RC12_MAX parameter; RC13_MAX parameter; RC14_MAX parameter; RC15_MAX parameter; RC16_MAX parameter; RC17_MAX parameter; RC18_MAX parameter; RC1_REV parameter; RC2_REV parameter; RC3_REV parameter; RC4_REV parameter; RC5_REV parameter; RC6_REV parameter; RC7_REV parameter; RC8_REV parameter; RC9_REV parameter; RC10_REV parameter; RC11_REV parameter; RC12_REV parameter; RC13_REV parameter; RC14_REV parameter; RC15_REV parameter; RC16_REV parameter; RC17_REV parameter; RC18_REV parameter; RC1_DZ parameter; RC2_DZ parameter; RC3_DZ parameter; RC4_DZ parameter; RC5_DZ parameter; RC6_DZ parameter; RC7_DZ parameter; RC8_DZ parameter; RC9_DZ parameter; RC10_DZ parameter; RC11_DZ parameter; RC12_DZ parameter; RC13_DZ parameter; RC14_DZ parameter; RC15_DZ parameter; RC16_DZ parameter; RC17_DZ parameter; RC18_DZ parameter; RC_INPUT_LOWEST_MIN_US constant int16 =uint64(500); RC_INPUT_HIGHEST_MAX_US constant int16 =uint64(2500); COM_ARM_MAG_STR parameter; COM_ARM_EKF_HGT parameter; COM_ARM_EKF_VEL parameter; COM_ARM_EKF_POS parameter; COM_ARM_EKF_YAW parameter; angular_velocity input Bus: px4_vehicle_angular_velocity; POSVEL_PROBATION_MAX constant uint64 =uint64(100*1e+6); COM_VEL_FS_EVH parameter; geofence_result input Bus: px4_geofence_result; geofence_warning_action_on_ local boolean =false; manual_control_setpoint input Bus: px4_manual_control_setpoint; COM_RC_LOSS_T parameter; COM_RC_ARM_HYST parameter; COM_ARM_SWISBTN parameter
  events: EVT_DISARM local FUNCTION_CALL_EVENT; EVT_AUTO_DISARM_LAND local FUNCTION_CALL_EVENT; EVT_AUTO_DISARM_PREFLIGHT local FUNCTION_CALL_EVENT; EVT_KILL_SWITCH local FUNCTION_CALL_EVENT; EVT_LOCKDOWN local FUNCTION_CALL_EVENT; EVT_SAFETY_BUTTON local FUNCTION_CALL_EVENT; EVT_ARM_RC_STICK local FUNCTION_CALL_EVENT; EVT_DISARM_RC_STICK local FUNCTION_CALL_EVENT
  function ret = is_vtol_tailsitter(current_status):
    | function ret = is_vtol_tailsitter(current_status)
    | 
    | ret = (current_status.system_type == VEHICLE_TYPE_VTOL_DUOROTOR || ...
    |     current_status.system_type == VEHICLE_TYPE_VTOL_QUADROTOR);
    | 
    | end
  function ret = is_rotary_wing(current_status):
    | function ret = is_rotary_wing(current_status)
    | 
    | ret = is_multirotor(current_status) || ...
    |     (current_status.system_type == VEHICLE_TYPE_HELICOPTER) || ...
    |     (current_status.system_type == VEHICLE_TYPE_COAXIAL);
    | 
    | end
  function ret = is_vtol(current_status):
    | function ret = is_vtol(current_status)
    | 
    | ret = (current_status.system_type == VEHICLE_TYPE_VTOL_DUOROTOR || ...
    |     current_status.system_type == VEHICLE_TYPE_VTOL_QUADROTOR || ...
    |     current_status.system_type == VEHICLE_TYPE_VTOL_TILTROTOR || ...
    |     current_status.system_type == VEHICLE_TYPE_VTOL_RESERVED2 || ...
    |     current_status.system_type == VEHICLE_TYPE_VTOL_RESERVED3 || ...
    |     current_status.system_type == VEHICLE_TYPE_VTOL_RESERVED4 || ...
    |     current_status.system_type == VEHICLE_TYPE_VTOL_RESERVED5);
    | 
    | end
  function commander_init:
    | function commander_init()
    | 
    | actuator_armed_out_ = actuator_armed;
    | battery_status_out_ = battery_status;
    | home_position_out_ = home_position;
    | control_mode_out_ = px4_vehicle_control_mode_zero();
    | internal_state_out_ = px4_commander_state_zero();
    | 
    | % default landed
    | land_detector_.landed = true;
    | 
    | % XXX for now just set sensors as initialized
    | vehicle_status_flags_out_.condition_system_sensors_initialized = true;
    | 
    | % We want to accept RC inputs as default
    | vehicle_status_out_.rc_input_mode = uint8(PX4_VEHICLE_STATUS.RC_IN_MODE_DEFAULT);
    | vehicle_status_out_.nav_state = uint8(PX4_VEHICLE_STATUS.NAVIGATION_STATE_MANUAL);
    | vehicle_status_out_.nav_state_timestamp = uint64(getSimulationTime*1e+6);
    | vehicle_status_out_.arming_state = uint8(PX4_VEHICLE_STATUS.ARMING_STATE_INIT);
    | 
    | % mark all signals lost as long as they haven't been found
    | vehicle_status_out_.rc_signal_lost = true;
    | vehicle_status_out_.data_link_lost = true;
    | 
    | % vehicle_status_flags
    | vehicle_status_flags_out_.offboard_control_signal_lost = true;
    | vehicle_status_flags_out_.condition_power_input_valid = true;
    | vehicle_status_flags_out_.rc_calibration_valid = true;
    | 
    | % default for vtol is rotary wing
    | vtol_status_.vtol_in_rw_mode = true;
    | 
    | % record boot time (in us)
    | boot_timestamp_ = uint64(getSimulationTime*1e+6);
    | 
    | % initial paramsmeter time
    | last_lpos_fail_time_us_ = boot_timestamp_;
    | last_gpos_fail_time_us_ = boot_timestamp_;
    | last_lvel_fail_time_us_ = boot_timestamp_;
    | 
    | end
  function mission_init:
    | function mission_init()
    | 
    | % init mission state, do it here to allow navigator to use stored mission even if mavlink failed to start
    | % there need to publish "mission_s topic" !!!
    | 
    | end
  function buzzer_init:
    | function buzzer_init()
    | 
    | tune_durations_(uint8(PX4_TUNE_CONTROL.TUNE_ID_NOTIFY_POSITIVE)) = 800000;
    | tune_durations_(uint8(PX4_TUNE_CONTROL.TUNE_ID_NOTIFY_NEGATIVE)) = 900000;
    | tune_durations_(uint8(PX4_TUNE_CONTROL.TUNE_ID_NOTIFY_NEUTRAL)) = 500000;
    | tune_durations_(uint8(PX4_TUNE_CONTROL.TUNE_ID_ARMING_WARNING)) = 3000000;
    | tune_durations_(uint8(PX4_TUNE_CONTROL.TUNE_ID_HOME_SET)) = 800000;
    | tune_durations_(uint8(PX4_TUNE_CONTROL.TUNE_ID_BATTERY_WARNING_FAST)) = 800000;
    | tune_durations_(uint8(PX4_TUNE_CONTROL.TUNE_ID_BATTERY_WARNING_SLOW)) = 800000;
    | tune_durations_(uint8(PX4_TUNE_CONTROL.TUNE_ID_SINGLE_BEEP)) = 300000;
    | % tune_control_pub = orb_advertise_queue(ORB_ID(tune_control), &tune_control, tune_control_s::ORB_QUEUE_LENGTH);
    | 
    | end
  function led_init:
    | function led_init()
    | 
    | blink_msg_end = 0;
    | led_control_out_.led_mask = 0xff;
    | led_control_out_.mode = uint8(PX4_LED_CONTROL.MODE_OFF);
    | led_control_out_.priority = uint8(0);
    | led_control_out_.timestamp = uint64(getSimulationTime * 1e+6);
    | 
    | % led_control_pub = orb_advertise_queue(ORB_ID(led_control), &led_control, led_control_s::ORB_QUEUE_LENGTH);
    | %
    | % /* first open normal LEDs */
    | % fd_leds = px4_open(LED0_DEVICE_PATH, O_RDWR);
    | %
    | % if (fd_leds < 0) {
    | %     // there might not be an LED available, so don't make this an error
    | %     PX4_INFO("LED: open %s failed (%i)", LED0_DEVICE_PATH, errno);
    | %     return -errno;
    | %     }
    | %
    | %     /* the green LED is only available on FMUv5 */
    | %     px4_ioctl(fd_leds, LED_ON, LED_GREEN);
    | %
    | %     /* the blue LED is only available on AeroCore but not FMUv2 */
    | %     px4_ioctl(fd_leds, LED_ON, LED_BLUE);
    | %
    | %     /* switch blue off */
    | %         led_off(LED_BLUE);
    | %
    | %         /* we consider the amber led mandatory */
    | %         if (px4_ioctl(fd_leds, LED_ON, LED_AMBER)) {
    | %             PX4_WARN("Amber LED: ioctl fail");
    | %             return PX4_ERROR;
    | %             }
    | %
    | %             /* switch amber off */
    | %                 led_off(LED_AMBER);
    | 
    | end
  function vehicle_type_init:
    | function vehicle_type_init()
    | 
    | vehicle_status_out_.system_type = uint8(MAV_TYPE);
    | 
    | if is_rotary_wing(vehicle_status_out_) || is_vtol(vehicle_status_out_)
    |     vehicle_status_out_.vehicle_type = uint8(PX4_VEHICLE_STATUS.VEHICLE_TYPE_ROTARY_WING);
    | elseif is_fixed_wing(vehicle_status_out_)
    |     vehicle_status_out_.vehicle_type = uint8(PX4_VEHICLE_STATUS.VEHICLE_TYPE_FIXED_WING);
    | elseif is_ground_rover(vehicle_status_out_)
    |     vehicle_status_out_.vehicle_type = uint8(PX4_VEHICLE_STATUS.VEHICLE_TYPE_ROVER);
    | else
    |     vehicle_status_out_.vehicle_type = uint8(PX4_VEHICLE_STATUS.VEHICLE_TYPE_UNKNOWN);
    | end
    | 
    | vehicle_status_out_.is_vtol = is_vtol(vehicle_status_out_);
    | vehicle_status_out_.is_vtol_tailsitter = is_vtol_tailsitter(vehicle_status_out_);
    | vehicle_status_out_.system_id = uint8(MAV_SYS_ID);
    | 
    | end
  function arm_auth_init:
    | function arm_auth_init()
    | 
    | timeout = single(0.0);
    | timeout = COM_ARM_AUTH_TO;
    | param_com_arm_auth_timout_ = uint64(timeout*1e+6);
    | 
    | auth_method = int32(PX4_ARM_AUTH_METHODS.ARM_AUTH_METHOD_ARM_REQ);
    | auth_method = COM_ARM_AUTH_MET;
    | 
    | % 如果是两步解锁
    | if (auth_method >= 0) && (auth_method < int32(PX4_ARM_AUTH_METHODS.ARM_AUTH_METHOD_LAST))
    |     param_com_arm_auth_method_ = auth_method;
    | else
    |     param_com_arm_auth_method_ = int32(PX4_ARM_AUTH_METHODS.ARM_AUTH_METHOD_ARM_REQ);
    | end
    | 
    | param_com_arm_auth_id_ = COM_ARM_AUTH_ID;
    | 
    | % system_id = status_.system_id;
    | % command_ack_sub = orb_subscribe(ORB_ID(vehicle_command_ack));
    | % mavlink_log_pub = mav_log_pub;
    | 
    | end
  function com_params_update:
    | function com_params_update
    | 
    | % enable avoidance flags
    | vehicle_status_flags_out_.avoidance_system_required = boolean(COM_OBS_AVOID);
    | 
    | if hasChanged(params_update.timestamp) || param_init_forced_
    | 
    |     % parameters that can only be modified in unlocked state
    |     if ~actuator_armed.armed
    |         is_rotary = is_rotary_wing(vehicle_status_out_) || (is_vtol(vehicle_status_out_) && vtol_status.vtol_in_rw_mode);
    |         is_fixed = is_fixed_wing(vehicle_status_out_) ||  (is_vtol(vehicle_status_out_) && ~vtol_status.vtol_in_rw_mode);
    |         is_ground = is_ground_rover(vehicle_status_out_);
    |     end
    | 
    |     % disable manual override for all systems that rely on electronic stabilization
    |     % e.g.For the vtol, the aircraft interior will judge the current status (rotor or fixed wing) by itself.
    |     % At this time, the internal judgment status will override the manually set status
    |     if is_rotary
    |         vehicle_status_out_.vehicle_type = uint8(PX4_VEHICLE_STATUS.VEHICLE_TYPE_ROTARY_WING);
    |     elseif is_fixed
    |         vehicle_status_out_.vehicle_type = uint8(PX4_VEHICLE_STATUS.VEHICLE_TYPE_FIXED_WING);
    |     elseif is_ground
    |         vehicle_status_out_.vehicle_type = uint8(PX4_VEHICLE_STATUS.VEHICLE_TYPE_ROVER);
    |     end
    | 
    |     vehicle_status_out_.is_vtol = is_vtol(vehicle_status_out_);
    |     vehicle_status_out_.is_vtol_tailsitter = is_vtol_tailsitter(vehicle_status_out_);
    | 
    |     % check and update system / component ID
    |     vehicle_status_out_.system_id = uint8(MAV_SYS_ID);
    |     vehicle_status_out_.component_id = uint8(MAV_COMP_ID);
    |     get_circuit_breaker_params();
    |     g_status_changed = true;
    | 
    |     % parameters that can be modified without being affected by the unlocking status
    |     vehicle_status_flags_out_.avoidance_system_required = boolean(COM_OBS_AVOID);
    |     vehicle_status_out_.rc_input_mode = uint8(COM_RC_IN_MODE);
    | 
    |     % arming conditions
    |     arm_requirements_.arm_authorization = boolean(COM_ARM_AUTH_REQ);
    |     arm_requirements_.esc_check = boolean(COM_ARM_CHK_ESCS);
    |     arm_requirements_.global_position = ~boolean(COM_ARM_WO_GPS);
    |     arm_requirements_.mission = boolean(COM_ARM_MIS_REQ);
    |     arm_requirements_.geofence = (GF_ACTION > PX4_GEOFENCE_RESULT.GF_ACTION_NONE);
    | 
    |     % flight mode slots
    |     flight_mode_slots_ = [COM_FLTMODE1, COM_FLTMODE2, COM_FLTMODE3, COM_FLTMODE4, COM_FLTMODE5, COM_FLTMODE6];
    | 
    |     % Check the airmode: Yaw airmode needs to use the unlock switch
    |     if (MC_AIRMODE == 2) && (RC_MAP_ARM_SW == 0)
    |         % airmode = 1; % change to roll/pitch airmode
    |         % param_set(param_airmode, &airmode);
    |         sprintf("Yaw Airmode requires the use of an Arm Switch");
    |     end
    |     param_init_forced_ = false;
    | 
    | end
    | 
    | end
  function ret = magnetometerCheck(instance, optional_mag, is_report_mag_fail):
    | function ret = magnetometerCheck(instance, optional_mag, is_report_mag_fail)
    | 
    | exists = true; % 此处暂时写为true, 后续结合嵌入式端判断mag是否存在
    | device_id = -1;
    | calibration_valid = false;
    | index = 0;
    | is_mag_fault = false;
    | 
    | if exists
    | 
    |     valid = (sensor_mag(instance).device_id ~= 0) && (sensor_mag(instance).timestamp ~= 0);
    | 
    |     if ~valid && is_report_mag_fail
    |         sprintf("mavlink_log_critical, Preflight Fail: no valid data from Compass.");
    |     end
    | 
    |     device_id = sensor_mag(instance).device_id;
    | 
    |     % 硬件在环仿真，忽略磁力计校准结果
    |     if vehicle_status_out_.hil_state == PX4_VEHICLE_STATUS.HIL_STATE_ON
    |         calibration_valid = true;
    |     else
    |         calibration_valid = true; % 此处暂时写为成功(calibration::FindCalibrationIndex("MAG", device_id) >= 0);
    |     end
    | 
    |     if ~calibration_valid && is_report_mag_fail
    |         sprintf("mavlink_log_citical, Preflight Fail: Compass uncalibrated.");
    |     end
    | 
    |     % for index = 1:max_optional_mag_count
    |     %
    |     % end
    | 
    |     if is_mag_fault && is_report_mag_fail
    |         sprintf("mavlink_log_citical, Preflight Fail: Compass %f fault.");
    |     end
    | 
    | else
    | 
    |     if ~optional_mag && is_report_mag_fail
    |         sprintf("mavlink_log_citical, Preflight Fail: Compass %f missing.");
    |     end
    | 
    | end
    | 
    | success = calibration_valid && ~is_mag_fault;
    | 
    | if instance == 0
    |     set_health_flags(SUBSYSTEM_TYPE_MAG, exists, ~optional_mag, success, vehicle_status_out_);
    | elseif instance == 1
    |     set_health_flags(SUBSYSTEM_TYPE_MAG, exists, ~optional_mag, success, vehicle_status_out_);
    | end
    | 
    | ret = success;
    | 
    | end
  function ret = magConsistencyCheck(report_status):
    | function ret = magConsistencyCheck(report_status)
    | 
    | pass = false; % flag for result of checks
    | 
    | % Use the difference between sensors to detect a bad calibration, orientation or magnetic interference.
    | % If a single sensor is fitted, the value being checked will be zero so this check will always pass.
    | angle_difference_limit_deg = single(90);
    | angle_difference_limit_deg = single(COM_ARM_MAG_ANG);
    | 
    | pass = pass || (angle_difference_limit_deg < 0); % disabled, pass check
    | pass = pass || (sensors.mag_inconsistency_angle < deg2rad(angle_difference_limit_deg));
    | 
    | if ~pass && report_status
    |     sprintf("mavlink_log_critical, Preflight Fail: Compasses %.4f deg inconsistent", rad2deg(sensors.mag_inconsistency_angle))
    |     sprintf("mavlink_log_critical, Please check orientations and recalibrate");
    |     % set_health_flags(uint64_t subsystem_type, bool present, bool enabled, bool ok, vehicle_status_s &status)
    |     % 第二个参数 present = status.onboard_control_sensors_present & (uint32_t)subsystem_type
    |     % 第三个参数enable = status.onboard_control_sensors_enabled & (uint32_t)subsystem_type
    |     set_health_flags(SUBSYSTEM_TYPE_MAG, ...
    |         bitand(vehicle_status_out_.onboard_control_sensors_present, SUBSYSTEM_TYPE_MAG), ...
    |         ~bitand(vehicle_status_out_.onboard_control_sensors_enabled, SUBSYSTEM_TYPE_MAG), ...
    |         false, ...
    |         vehicle_status_out_);
    |     set_health_flags(SUBSYSTEM_TYPE_MAG2, ...
    |         bitand(vehicle_status_out_.onboard_control_sensors_present, SUBSYSTEM_TYPE_MAG), ...
    |         ~bitand(vehicle_status_out_.onboard_control_sensors_enabled, SUBSYSTEM_TYPE_MAG), ...
    |         false, ...
    |         vehicle_status_out_);
    | end
    | 
    | ret = true;
    | 
    | end
  function ret = accelerometerCheck(instance, optional_accel, is_report_accel_fail):
    | function ret = accelerometerCheck(instance, optional_accel, is_report_accel_fail)
    | 
    | exists = true; % 此处暂时写为true, 后续结合嵌入式端判断accel是否存在
    | device_id = -1;
    | calibration_valid = false;
    | valid = true;
    | index = 0;
    | 
    | if exists
    |     %% 加表存在
    |     valid = (sensor_accel(instance).device_id ~= 0) && (sensor_accel(instance).timestamp ~= 0);
    | 
    |     if ~valid && is_report_accel_fail
    |         sprintf("mavlink_log_critical, Preflight Fail: no valid data from Accel %u", instance);
    |     end
    | 
    |     device_id = sensor_accel(instance).device_id;
    | 
    |     % 硬件在环仿真，忽略加表校准结果
    |     if vehicle_status_out_.hil_state == PX4_VEHICLE_STATUS.HIL_STATE_ON
    |         calibration_valid = true;
    |     else
    |         calibration_valid = true; % 此处暂时写为成功(calibration::FindCalibrationIndex("ACC", device_id) >= 0);
    |     end
    | 
    |     if ~calibration_valid && is_report_accel_fail
    |         sprintf("mavlink_log_citical, Preflight Fail: Accel %u uncalibrated", instance);
    |     else
    |         accel_magnitude = sqrt(sensor_accel(instance).x * sensor_accel(instance).x + ...
    |             sensor_accel(instance).y * sensor_accel(instance).y + ...
    |             sensor_accel(instance).z * sensor_accel(instance).z);
    |         if accel_magnitude < 4.0 || accel_magnitude > 15.0 % m/s^2
    |             if is_report_accel_fail
    |                 sprintf("mavlink_log_critical, Preflight Fail: Accel Range, hold still on arming");
    |             end
    |             % this is fatal
    |             valid = false;
    |         end
    |     end
    | 
    | else
    |     %% 加表不存在
    |     if ~optional_accel && is_report_accel_fail
    |         sprintf("mavlink_log_citical, Preflight Fail: Accel Sensor %u missing", instance);
    |     end
    | 
    | end
    | 
    | ret = calibration_valid && valid;
    | 
    | end
  function ret = gyroCheck(instance, optional_gyro, is_report_gyro_fail):
    | function ret = gyroCheck(instance, optional_gyro, is_report_gyro_fail)
    | 
    | exists = true; % 此处暂时写为true, 后续结合嵌入式端判断gyro是否存在
    | device_id = -1;
    | calibration_valid = false;
    | valid = true;
    | index = 0;
    | 
    | if exists
    |     %% 陀螺仪存在
    |     valid = (sensor_gyro(instance).device_id ~= 0) && (sensor_gyro(instance).timestamp ~= 0);
    | 
    |     if ~valid && is_report_gyro_fail
    |         sprintf("mavlink_log_critical, Preflight Fail: no valid data from Gyro %u", instance);
    |     end
    | 
    |     device_id = sensor_gyro(instance).device_id;
    | 
    |     % 硬件在环仿真，忽略加表校准结果
    |     if vehicle_status_out_.hil_state == PX4_VEHICLE_STATUS.HIL_STATE_ON
    |         calibration_valid = true;
    |     else
    |         calibration_valid = true; % 此处暂时写为成功(calibration::FindCalibrationIndex("GYRO", device_id) >= 0);
    |     end
    | 
    |     if ~calibration_valid && is_report_gyro_fail
    |         sprintf("mavlink_log_citical, Preflight Fail: sensor_gyro %u uncalibrated", instance);
    |     end
    | 
    | else
    |     %% 陀螺仪不存在
    |     if ~optional_gyro && is_report_gyro_fail
    |         sprintf("mavlink_log_citical, Preflight Fail: Gyro Sensor %u missing", instance);
    |     end
    | 
    | end
    | 
    | ret = calibration_valid && valid;
    | 
    | end
  function ret = baroCheck(instance, optional_baro, is_report_baro_fail):
    | function ret = baroCheck(instance, optional_baro, is_report_baro_fail)
    | 
    | exists = true; % 此处暂时写为true, 后续结合嵌入式端判断accel是否存在
    | device_id = -1;
    | valid = false;
    | index = 0;
    | 
    | if exists
    |     %% 气压计存在
    |     valid = (sensor_gyro(instance).device_id ~= 0) && (sensor_gyro(instance).timestamp ~= 0);
    | 
    |     if ~valid && is_report_baro_fail
    |         sprintf("mavlink_log_critical, Preflight Fail: no valid data from Baro %u", instance);
    |     end
    | 
    | else
    |     %% 气压计不存在
    |     if ~optional_baro && is_report_baro_fail
    |         sprintf("mavlink_log_citical, Preflight Fail: Baro Sensor %u missing", instance);
    |     end
    | 
    | end
    | 
    | if instance == 0
    |     set_health_flags(SUBSYSTEM_TYPE_ABSPRESSURE, ...
    |         exists, ...
    |         ~optional_baro, ...
    |         valid, ...
    |         vehicle_status_out_);
    | end
    | 
    | ret = valid;
    | 
    | end
  function ret = imuConsistencyCheck(report_status):
    | function ret = imuConsistencyCheck(report_status)
    | 
    | accel_test_limit = single(1.0);
    | accel_test_limit = COM_ARM_IMU_ACC;
    | 
    | gyro_test_limit = single(1.0);
    | gyro_test_limit = COM_ARM_IMU_GYR;
    | 
    | % Use the difference between IMU's to detect a bad calibration.
    | % If a single IMU is fitted, the value being checked will be zero so this check will always pass.
    | for i = 1:max_optional_accel_count
    |     if sensors_status_imu.accel_device_ids(i) ~= 0
    |         if sensors_status_imu.accel_device_ids(i) == sensors_status_imu.accel_device_id_primary
    |             set_health_flags_healthy(SUBSYSTEM_TYPE_ACC, sensors_status_imu.accel_healthy(i), vehicle_status_out_);
    |         else
    |             set_health_flags_healthy(SUBSYSTEM_TYPE_ACC2, sensors_status_imu.accel_healthy(i), vehicle_status_out_);
    |         end
    | 
    |         accel_inconsistency_m_s_s = sensors_status_imu.accel_inconsistency_m_s_s(i);
    | 
    |         if accel_inconsistency_m_s_s > accel_test_limit
    |             if report_status
    |                 sprintf("mavlink_log_critical, Preflight Fail: Accel %u inconsistent - Check Cal", i);
    |                 if sensors_status_imu.accel_device_ids(i) == sensors_status_imu.accel_device_id_primary
    |                     set_health_flags_healthy(SUBSYSTEM_TYPE_ACC, false, vehicle_status_out_);
    |                 else
    |                     set_health_flags_healthy(SUBSYSTEM_TYPE_ACC2, false, vehicle_status_out_);
    |                 end
    |             end
    | 
    |             ret = false;
    |             return
    | 
    |         elseif (accel_inconsistency_m_s_s > accel_test_limit * 0.8) && report_status
    |             sprintf("mavlink_log_info, Preflight Advice: Accel %u inconsistent - Check Cal", i);
    |         end
    |     end
    | end
    | 
    | % Fail if gyro difference greater than 5 deg/sec and notify if greater than 2.5 deg/sec
    | for i = 1:max_optional_gyro_count
    |     if sensors_status_imu.gyro_device_ids(i) ~= 0
    |         if sensors_status_imu.gyro_device_ids(i) == sensors_status_imu.gyro_device_id_primary
    |             set_health_flags_healthy(SUBSYSTEM_TYPE_GYRO, sensors_status_imu.accel_healthy(i), vehicle_status_out_);
    |         else
    |             set_health_flags_healthy(SUBSYSTEM_TYPE_GYRO2, sensors_status_imu.accel_healthy(i), vehicle_status_out_);
    |         end
    | 
    |         gyro_inconsistency_rad_s = sensors_status_imu.gyro_inconsistency_rad_s(i);
    | 
    |         if gyro_inconsistency_rad_s > gyro_test_limit
    |             if report_status
    |                 sprintf("mavlink_log_critical, Preflight Fail: Gyro %u inconsistent - Check Cal", i);
    | 
    |                 if sensors_status_imu.gyro_device_ids(i) == sensors_status_imu.gyro_device_id_primary
    |                     set_health_flags_healthy(SUBSYSTEM_TYPE_GYRO, false, vehicle_status_out_);
    |                 else
    |                     set_health_flags_healthy(SUBSYSTEM_TYPE_GYRO2, false, vehicle_status_out_);
    |                 end
    | 
    |                 ret = false;
    |                 return
    | 
    |             elseif (gyro_inconsistency_rad_s > gyro_test_limit * 0.5) && report_status
    |                 sprintf("mavlink_log_info, Preflight Advice: Gyro %u inconsistent - Check Cal", i);
    |             end
    |         end
    |     end
    | end
    | 
    | ret = true;
    | 
    | end
  function ret = airspeedCheck(optional_aspd, report_failures, ...:
    | function ret = airspeedCheck(optional_aspd, report_failures, ...
    |     prearm, max_aspd_check_en, arming_max_aspd_allowed)
    | 
    | present = true;
    | success = true;
    | ret = true;
    | 
    | %% Check if Airspeed Selector is up and running.
    | if (uint64(getSimulationTime*1e+6) - airspeed_validated.timestamp) > 1e+6
    |     if report_failures && ~optional_aspd
    |         sprintf("mavlink_log_critical, Preflight Fail: Airspeed Selector module down.");
    |     end
    |     present = false;
    |     success = false;
